simulink model "Impedance_Control"  (R2021b)
settings: Solver=VariableStepAuto  StartTime=0.0  StopTime=10  RelTol=1e-3
undefined symbols (not defined in the file or in its folder): Dm, Km, q_dq_init
(part 2 of 3)

== matlab function Impedance_Control/C ==
  data: q input; C output; dq input
function C = C(q,dq)
%C_fun
%    C = C_fun(Q1,Q2,Q3,Q4,Q5,Q6,DQ1,DQ2,DQ3,DQ4,DQ5,DQ6)

%    This function was generated by the Symbolic Math Toolbox version 9.0.
%    28-Mar-2022 14:37:35

q1 = q(1);
q2 = q(2);
q3 = q(3);
q4 = q(4);
q5 = q(5);
q6 = q(6);

dq1 = dq(1);
dq2 = dq(2);
dq3 = dq(3);
dq4 = dq(4);
dq5 = dq(5);
dq6 = dq(6);

t2 = cos(q1);
t3 = cos(q2);
t4 = cos(q4);
t5 = cos(q5);
t6 = cos(q6);
t7 = sin(q1);
t8 = sin(q2);
t9 = sin(q4);
t10 = sin(q5);
t11 = sin(q6);
t12 = dq1.^2;
t13 = dq2.^2;
t14 = dq4.^2;
t15 = dq5.^2;
t16 = dq6.^2;
t17 = q2.*2.0;
t18 = q3.^2;
t291 = q3-5.6e-3;
t555 = q3-1.56e-2;
t19 = cos(t17);
t20 = t3.^2;
t21 = t4.^2;
t22 = sin(t17);
t23 = t8.^2;
t24 = t9.^2;
t25 = dq2.*t4;
t26 = dq3.*t8;
t27 = dq2.*t9;
t28 = t2.*t4;
t29 = t3.*t5;
t31 = t2.*t9;
t32 = t4.*t7;
t33 = t3.*t10;
t34 = t5.*t8;
t35 = t7.*t9;
t36 = t8.*t10;
t38 = dq1.*t2.*t3;
t40 = dq3.*t2.*t3;
t41 = dq1.*t3.*t4;
t45 = dq4.*t3.*t4;
t47 = dq1.*t3.*t7;
t48 = dq2.*t2.*t8;
t51 = dq3.*t3.*t7;
t52 = dq1.*t3.*t9;
t59 = dq4.*t3.*t9;
t60 = dq4.*t4.*t8;
t63 = dq2.*t7.*t8;
t68 = dq4.*t8.*t9;
t70 = dq2.*dq3.*t3.*2.0;
t74 = t8.*t9.*t11;
t80 = t3.*t4.*t6;
t93 = t3.*t4.*t11;
t94 = t3.*t6.*t9;
t107 = t3.*t9.*t11;
t108 = t6.*t8.*t9;
t250 = t3.*t4.*t13;
t252 = t3.*t4.*t14;
t258 = t3.*t9.*t13;
t262 = t3.*t9.*t14;
t277 = t8.*t13.*1.56e+2;
t574 = dq2.*dq3.*t3.*2.0e+4;
t615 = t2.*t3.*t12.*1.56e+2;
t616 = t2.*t3.*t13.*1.56e+2;
t627 = t3.*t7.*t12.*1.56e+2;
t628 = t3.*t7.*t13.*1.56e+2;
t675 = q3.*t8.*t13.*1.0e+4;
t847 = dq2.*t3.*t291;
t928 = q3.*t2.*t3.*t12.*1.0e+4;
t929 = q3.*t2.*t3.*t13.*1.0e+4;
t935 = q3.*t3.*t7.*t12.*1.0e+4;
t936 = q3.*t3.*t7.*t13.*1.0e+4;
t945 = dq2.*t3.*t555;
t1137 = t8.*t13.*t291;
t1202 = t8.*t13.*t555;
t1234 = t2.*t3.*t12.*t291;
t1235 = t2.*t3.*t13.*t291;
t1241 = t3.*t7.*t12.*t291;
t1242 = t3.*t7.*t13.*t291;
t1250 = t2.*t3.*t12.*t555;
t1251 = t2.*t3.*t13.*t555;
t1255 = t3.*t7.*t12.*t555;
t1256 = t3.*t7.*t13.*t555;
t30 = dq4.*t27;
t37 = dq4.*t25;
t39 = dq1.*t28;
t42 = t3.*t25;
t43 = dq2.*t29;
t44 = dq4.*t28;
t46 = dq5.*t29;
t49 = dq1.*t31;
t50 = dq1.*t32;
t53 = t3.*t27;
t54 = t8.*t25;
t55 = dq2.*t33;
t56 = dq2.*t34;
t57 = dq4.*t31;
t58 = dq4.*t32;
t61 = dq5.*t33;
t62 = dq5.*t34;
t64 = dq1.*t35;
t65 = t8.*t27;
t66 = dq2.*t36;
t67 = dq4.*t35;
t69 = dq5.*t36;
t71 = t8.*t35;
t72 = t7.*t36;
t73 = t10.*t35;
t75 = t11.*t36;
t76 = dq4.*t41;
t77 = t2.*t29;
t78 = t5.*t28;
t79 = t4.*t29;
t81 = t6.*t29;
t83 = dq4.*t52;
t84 = t8.*t28;
t85 = t2.*t33;
t86 = t2.*t34;
t87 = t7.*t29;
t88 = t10.*t28;
t89 = t5.*t31;
t90 = t5.*t32;
t91 = t4.*t33;
t92 = t4.*t34;
t95 = t11.*t29;
t96 = t6.*t34;
t98 = t8.*t31;
t99 = t8.*t32;
t100 = t2.*t36;
t101 = t7.*t33;
t102 = t7.*t34;
t103 = t10.*t31;
t104 = t10.*t32;
t105 = t5.*t35;
t106 = t4.*t36;
t109 = t11.*t34;
t110 = t6.*t36;
t111 = -t70;
t119 = t25.*t29;
t125 = t6.*t45;
t127 = dq6.*t80;
t147 = t25.*t33;
t148 = t25.*t34;
t161 = dq4.*t9.*t29;
t165 = t11.*t45;
t166 = t6.*t59;
t167 = t6.*t60;
t173 = dq6.*t93;
t174 = dq6.*t94;
t195 = t25.*t36;
t196 = t27.*t34;
t208 = dq4.*t9.*t33;
t209 = dq4.*t9.*t34;
t213 = t11.*t59;
t214 = t11.*t60;
t220 = dq6.*t107;
t221 = dq6.*t108;
t224 = -t40;
t233 = t27.*t36;
t237 = dq4.*t9.*t36;
t240 = dq6.*t74;
t242 = -t51;
t243 = -t52;
t244 = -t63;
t248 = -t68;
t249 = t12.*t28;
t251 = t14.*t28;
t253 = dq3.*t38.*2.0;
t256 = t12.*t31;
t257 = t12.*t32;
t259 = t13.*t34;
t260 = t14.*t31;
t261 = t14.*t32;
t263 = t15.*t34;
t264 = dq3.*t47.*2.0;
t265 = dq2.*t2.*t26.*2.0;
t270 = t12.*t35;
t271 = t13.*t36;
t272 = t14.*t35;
t273 = t15.*t36;
t274 = dq2.*t7.*t26.*2.0;
t279 = t38.*1.56e+2;
t280 = t47.*1.56e+2;
t281 = t48.*1.56e+2;
t282 = t63.*1.56e+2;
t283 = t28.*t29;
t285 = t28.*t33;
t286 = t28.*t34;
t287 = t29.*t32;
t288 = t3.*t6.*t31;
t292 = t28.*t36;
t293 = t31.*t34;
t294 = t32.*t33;
t295 = t32.*t34;
t296 = t3.*t11.*t31;
t297 = t3.*t6.*t35;
t299 = t6.*t9.*t33;
t305 = t31.*t36;
t306 = t32.*t36;
t307 = t34.*t35;
t308 = t3.*t11.*t35;
t309 = t9.*t11.*t33;
t315 = -t94;
t316 = t35.*t36;
t323 = -t277;
t466 = t25.*t38.*2.0;
t484 = t13.*t94;
t489 = t14.*t94;
t492 = t16.*t94;
t494 = t27.*t38.*2.0;
t525 = t13.*t107;
t531 = t14.*t107;
t533 = t16.*t107;
t535 = t27.*t47.*2.0;
t570 = dq1.*t48.*3.12e+2;
t573 = dq1.*t63.*3.12e+2;
t576 = dq6.*t6.*t28.*1.0e+2;
t583 = dq6.*t6.*t32.*1.0e+2;
t592 = t40.*1.0e+4;
t595 = t27+t41;
t596 = t51.*1.0e+4;
t634 = -t574;
t782 = dq3.*t38.*2.0e+4;
t787 = q3.*t38.*1.0e+4;
t788 = dq3.*t47.*2.0e+4;
t789 = dq2.*t2.*t26.*2.0e+4;
t790 = q3.*t47.*1.0e+4;
t791 = q3.*t48.*1.0e+4;
t792 = dq2.*t7.*t26.*2.0e+4;
t793 = q3.*t63.*1.0e+4;
t830 = dq1.*q3.*t48.*2.0e+4;
t834 = t47+t48;
t844 = dq1.*q3.*t63.*2.0e+4;
t880 = t11.*t16.*t28.*1.0e+2;
t904 = t11.*t16.*t32.*1.0e+2;
t968 = t11.*t27.*t38.*2.0e+2;
t991 = t11.*t27.*t47.*2.0e+2;
t1030 = t38.*t291;
t1031 = -t928;
t1032 = -t929;
t1035 = t47.*t291;
t1036 = t48.*t291;
t1037 = -t935;
t1038 = -t936;
t1043 = t63.*t291;
t1145 = t38.*t555;
t1148 = t47.*t555;
t1149 = t48.*t555;
t1152 = t63.*t555;
t1248 = t26+t847;
t1287 = -t1250;
t1288 = -t1251;
t1290 = -t1255;
t1291 = -t1256;
t1399 = t25.*1.0e-1;
t1402 = t27.*1.0e-1;
t1412 = t41.*1.0e-1;
t1415 = t52.*1.0e-1;
t82 = dq1.*t54;
t97 = dq1.*t65;
t112 = -t37;
t113 = t3.*t39;
t114 = dq1.*t77;
t115 = t2.*t42;
t116 = t2.*t43;
t117 = t5.*t39;
t118 = t3.*t44;
t120 = t2.*t46;
t121 = t5.*t44;
t122 = t6.*t43;
t123 = dq4.*t79;
t124 = dq5.*t78;
t126 = t4.*t46;
t128 = dq6.*t81;
t129 = t3.*t49;
t130 = t8.*t39;
t131 = t3.*t50;
t132 = dq1.*t85;
t133 = dq1.*t86;
t134 = dq1.*t87;
t135 = t2.*t53;
t136 = t2.*t54;
t137 = t7.*t42;
t138 = t2.*t55;
t139 = t2.*t56;
t140 = t7.*t43;
t141 = t10.*t39;
t142 = t5.*t49;
t143 = t5.*t50;
t144 = t3.*t57;
t145 = t8.*t44;
t146 = t3.*t58;
t149 = t2.*t61;
t150 = t2.*t62;
t151 = t7.*t46;
t152 = t6.*t53;
t153 = t6.*t54;
t154 = t10.*t44;
t155 = t5.*t57;
t156 = t5.*t58;
t157 = t11.*t43;
t158 = t6.*t55;
t159 = t6.*t56;
t160 = dq4.*t91;
t162 = dq5.*t88;
t163 = dq5.*t89;
t164 = dq5.*t90;
t168 = t4.*t61;
t169 = t9.*t46;
t170 = t4.*t62;
t171 = t6.*t61;
t172 = t6.*t62;
t175 = dq6.*t95;
t176 = dq6.*t96;
t177 = t8.*t49;
t178 = t3.*t64;
t179 = t8.*t50;
t180 = dq1.*t100;
t181 = dq1.*t101;
t182 = dq1.*t102;
t183 = t2.*t65;
t184 = t7.*t53;
t185 = t7.*t54;
t186 = t2.*t66;
t187 = t7.*t55;
t188 = t7.*t56;
t189 = t10.*t49;
t190 = t10.*t50;
t191 = t5.*t64;
t192 = t8.*t57;
t193 = t3.*t67;
t194 = t8.*t58;
t197 = t2.*t69;
t198 = t7.*t61;
t199 = t7.*t62;
t200 = t11.*t53;
t201 = t11.*t54;
t202 = t6.*t65;
t203 = t10.*t57;
t204 = t10.*t58;
t205 = t5.*t67;
t206 = t11.*t55;
t207 = t11.*t56;
t210 = dq5.*t103;
t211 = dq5.*t104;
t212 = dq5.*t105;
t215 = t9.*t61;
t216 = t4.*t69;
t217 = t11.*t61;
t218 = t11.*t62;
t219 = t6.*t69;
t222 = dq6.*t109;
t223 = dq6.*t110;
t225 = -t43;
t226 = -t46;
t227 = t8.*t64;
t228 = dq1.*t72;
t229 = t7.*t65;
t230 = t7.*t66;
t231 = t10.*t64;
t232 = t8.*t67;
t234 = t7.*t69;
t235 = t11.*t65;
t236 = t10.*t67;
t238 = dq5.*t73;
t239 = t11.*t69;
t241 = dq6.*t75;
t245 = -t64;
t246 = -t65;
t247 = -t67;
t254 = dq4.*t39.*2.0;
t255 = dq5.*t43.*2.0;
t266 = dq4.*t49.*2.0;
t267 = dq4.*t50.*2.0;
t268 = t8.*t37.*2.0;
t269 = dq5.*t55.*2.0;
t275 = dq4.*t64.*2.0;
t276 = t8.*t30.*2.0;
t278 = -t71;
t284 = t6.*t79;
t289 = t11.*t79;
t290 = t6.*t91;
t298 = t11.*t91;
t300 = t6.*t106;
t301 = -t253;
t303 = -t79;
t304 = -t81;
t310 = t4.*t75;
t311 = -t264;
t312 = -t265;
t313 = -t84;
t314 = -t87;
t318 = -t274;
t321 = -t105;
t322 = -t106;
t324 = t29.*t39;
t325 = t25.*t77;
t327 = t28.*t46;
t330 = t33.*t39;
t331 = t34.*t39;
t332 = t29.*t50;
t334 = t25.*t85;
t335 = t27.*t77;
t336 = t25.*t86;
t337 = t25.*t87;
t338 = t29.*t57;
t339 = t34.*t44;
t342 = t28.*t61;
t343 = t28.*t62;
t344 = t32.*t46;
t345 = t6.*t147;
t346 = t25.*t96;
t347 = dq6.*t288;
t349 = dq4.*t9.*t81;
t356 = t36.*t39;
t357 = t34.*t49;
t358 = t33.*t50;
t359 = t34.*t50;
t362 = t27.*t85;
t363 = t25.*t100;
t364 = t25.*t101;
t365 = t27.*t87;
t366 = t25.*t102;
t368 = t33.*t57;
t369 = t36.*t44;
t370 = t34.*t57;
t371 = t29.*t67;
t372 = t34.*t58;
t374 = t28.*t69;
t375 = t31.*t62;
t376 = t32.*t61;
t377 = t32.*t62;
t378 = t11.*t147;
t379 = t25.*t109;
t380 = t25.*t110;
t381 = dq6.*t296;
t382 = dq6.*t297;
t384 = dq4.*t9.*t95;
t385 = t6.*t208;
t390 = dq6.*t299;
t398 = -t119;
t403 = -t125;
t405 = -t127;
t407 = t36.*t49;
t408 = t36.*t50;
t409 = t34.*t64;
t411 = t27.*t101;
t412 = t25.*t72;
t415 = t36.*t57;
t416 = t33.*t67;
t417 = t36.*t58;
t418 = t34.*t67;
t419 = t31.*t69;
t420 = t32.*t69;
t421 = t35.*t62;
t422 = t25.*t75;
t423 = t27.*t110;
t424 = dq6.*t308;
t425 = t11.*t208;
t426 = dq4.*t9.*t110;
t427 = dq6.*t309;
t430 = -t165;
t431 = -t167;
t432 = -t174;
t433 = t36.*t64;
t435 = t36.*t67;
t436 = t35.*t69;
t437 = t27.*t75;
t438 = dq4.*t9.*t75;
t450 = -t233;
t453 = -t237;
t457 = -t280;
t458 = -t281;
t459 = -t282;
t460 = t12.*t77;
t461 = t13.*t77;
t462 = t13.*t79;
t463 = t15.*t77;
t464 = t14.*t79;
t465 = t15.*t79;
t467 = t2.*t3.*t37.*2.0;
t472 = dq6.*t125.*2.0;
t473 = t12.*t84;
t474 = t12.*t85;
t475 = t12.*t87;
t476 = t13.*t84;
t477 = t13.*t85;
t478 = t13.*t87;
t479 = t12.*t89;
t480 = t14.*t84;
t481 = t13.*t91;
t482 = t15.*t85;
t483 = t15.*t87;
t485 = t14.*t89;
t486 = t13.*t96;
t487 = t14.*t91;
t488 = t15.*t89;
t490 = t15.*t91;
t491 = t15.*t96;
t493 = t16.*t96;
t498 = t2.*t3.*t30.*2.0;
C = ft_1({dq1,dq2,dq3,dq4,dq5,dq6,q3,t10,t100,t101,t102,t103,t1030,t1031,t1032,t1035,t1036,t1037,t1038,t104,t1043,t105,t106,t107,t108,t109,t11,t110,t111,t112,t113,t1137,t114,t1145,t1148,t1149,t115,t1152,t116,t117,t118,t12,t120,t1202,t121,t122,t123,t1234,t1235,t124,t1241,t1242,t1248,t125,t126,t128,t1287,t1288,t129,t1290,t1291,t13,t130,t131,t132,t133,t134,t135,t136,t137,t138,t139,t1399,t14,t140,t1402,t141,t1412,t1415,t142,t143,t144,t145,t146,t147,t148,t149,t15,t150,t151,t152,t153,t154,t155,t156,t157,t158,t159,t16,t160,t161,t162,t163,t164,t165,t166,t168,t169,t170,t171,t172,t173,t175,t176,t177,t178,t179,t18,t180,t181,t182,t183,t184,t185,t186,t187,t188,t189,t19,t190,t191,t192,t193,t194,t195,t196,t197,t198,t199,t2,t20,t200,t201,t202,t203,t204,t205,t206,t207,t208,t209,t21,t210,t211,t212,t213,t214,t215,t216,t217,t218,t219,t22,t220,t221,t222,t223,t224,t225,t226,t227,t228,t229,t23,t230,t231,t232,t233,t234,t235,t236,t238,t239,t24,t240,t241,t242,t243,t244,t245,t246,t247,t248,t249,t25,t250,t251,t252,t253,t254,t255,t256,t257,t258,t259,t26,t260,t261,t262,t263,t264,t265,t266,t267,t268,t269,t270,t271,t272,t273,t274,t275,t276,t278,t279,t28,t283,t284,t285,t286,t287,t288,t289,t29,t290,t291,t292,t293,t294,t295,t296,t297,t298,t299,t3,t30,t300,t301,t303,t304,t305,t306,t307,t308,t309,t31,t310,t311,t312,t313,t314,t315,t316,t318,t32,t321,t322,t323,t324,t325,t33,t330,t331,t332,t334,t335,t336,t337,t338,t339,t34,t342,t343,t344,t345,t346,t347,t349,t35,t356,t357,t358,t359,t36,t362,t363,t364,t365,t366,t368,t369,t37,t370,t371,t372,t374,t375,t376,t377,t378,t379,t38,t380,t381,t382,t384,t385,t39,t390,t398,t4,t40,t403,t405,t407,t408,t409,t411,t412,t415,t417,t419,t42,t420,t421,t422,t423,t424,t425,t426,t427,t43,t430,t431,t432,t433,t435,t436,t437,t438,t44,t45,t450,t453,t457,t458,t459,t460,t461,t463,t466,t467,t47,t472,t473,t474,t475,t476,t477,t478,t479,t48,t480,t481,t482,t483,t485,t486,t487,t488,t49,t490,t491,t493,t494,t498,t5,t50,t51,t525,t53,t531,t533,t535,t54,t55,t555,t56,t57,t570,t573,t576,t58,t583,t59,t592,t595,t596,t6,t60,t61,t615,t616,t62,t627,t628,t63,t634,t64,t65,t66,t67,t675,t69,t7,t70,t71,t72,t73,t74,t75,t76,t77,t78,t782,t787,t788,t789,t79,t790,t791,t792,t793,t8,t80,t81,t82,t83,t830,t834,t84,t844,t847,t85,t86,t87,t88,t880,t89,t9,t90,t904,t91,t92,t93,t94,t945,t95,t96,t968,t97,t98,t99,t991});
end
function C = ft_1(ct)
dq1 = ct{1};
dq2 = ct{2};
dq3 = ct{3};
dq4 = ct{4};
dq5 = ct{5};
dq6 = ct{6};
q3 = ct{7};
t10 = ct{8};
t100 = ct{9};
t101 = ct{10};
t102 = ct{11};
t103 = ct{12};
t1030 = ct{13};
t1031 = ct{14};
t1032 = ct{15};
t1035 = ct{16};
t1036 = ct{17};
t1037 = ct{18};
t1038 = ct{19};
t104 = ct{20};
t1043 = ct{21};
t105 = ct{22};
t106 = ct{23};
t107 = ct{24};
t108 = ct{25};
t109 = ct{26};
t11 = ct{27};
t110 = ct{28};
t111 = ct{29};
t112 = ct{30};
t113 = ct{31};
t1137 = ct{32};
t114 = ct{33};
t1145 = ct{34};
t1148 = ct{35};
t1149 = ct{36};
t115 = ct{37};
t1152 = ct{38};
t116 = ct{39};
t117 = ct{40};
t118 = ct{41};
t12 = ct{42};
t120 = ct{43};
t1202 = ct{44};
t121 = ct{45};
t122 = ct{46};
t123 = ct{47};
t1234 = ct{48};
t1235 = ct{49};
t124 = ct{50};
t1241 = ct{51};
t1242 = ct{52};
t1248 = ct{53};
t125 = ct{54};
t126 = ct{55};
t128 = ct{56};
t1287 = ct{57};
t1288 = ct{58};
t129 = ct{59};
t1290 = ct{60};
t1291 = ct{61};
t13 = ct{62};
t130 = ct{63};
t131 = ct{64};
t132 = ct{65};
t133 = ct{66};
t134 = ct{67};
t135 = ct{68};
t136 = ct{69};
t137 = ct{70};
t138 = ct{71};
t139 = ct{72};
t1399 = ct{73};
t14 = ct{74};
t140 = ct{75};
t1402 = ct{76};
t141 = ct{77};
t1412 = ct{78};
t1415 = ct{79};
t142 = ct{80};
t143 = ct{81};
t144 = ct{82};
t145 = ct{83};
t146 = ct{84};
t147 = ct{85};
t148 = ct{86};
t149 = ct{87};
t15 = ct{88};
t150 = ct{89};
t151 = ct{90};
t152 = ct{91};
t153 = ct{92};
t154 = ct{93};
t155 = ct{94};
t156 = ct{95};
t157 = ct{96};
t158 = ct{97};
t159 = ct{98};
t16 = ct{99};
t160 = ct{100};
t161 = ct{101};
t162 = ct{102};
t163 = ct{103};
t164 = ct{104};
t165 = ct{105};
t166 = ct{106};
t168 = ct{107};
t169 = ct{108};
t170 = ct{109};
t171 = ct{110};
t172 = ct{111};
t173 = ct{112};
t175 = ct{113};
t176 = ct{114};
t177 = ct{115};
t178 = ct{116};
t179 = ct{117};
t18 = ct{118};
t180 = ct{119};
t181 = ct{120};
t182 = ct{121};
t183 = ct{122};
t184 = ct{123};
t185 = ct{124};
t186 = ct{125};
t187 = ct{126};
t188 = ct{127};
t189 = ct{128};
t19 = ct{129};
t190 = ct{130};
t191 = ct{131};
t192 = ct{132};
t193 = ct{133};
t194 = ct{134};
t195 = ct{135};
t196 = ct{136};
t197 = ct{137};
t198 = ct{138};
t199 = ct{139};
t2 = ct{140};
t20 = ct{141};
t200 = ct{142};
t201 = ct{143};
t202 = ct{144};
t203 = ct{145};
t204 = ct{146};
t205 = ct{147};
t206 = ct{148};
t207 = ct{149};
t208 = ct{150};
t209 = ct{151};
t21 = ct{152};
t210 = ct{153};
t211 = ct{154};
t212 = ct{155};
t213 = ct{156};
t214 = ct{157};
t215 = ct{158};
t216 = ct{159};
t217 = ct{160};
t218 = ct{161};
t219 = ct{162};
t22 = ct{163};
t220 = ct{164};
t221 = ct{165};
t222 = ct{166};
t223 = ct{167};
t224 = ct{168};
t225 = ct{169};
t226 = ct{170};
t227 = ct{171};
t228 = ct{172};
t229 = ct{173};
t23 = ct{174};
t230 = ct{175};
t231 = ct{176};
t232 = ct{177};
t233 = ct{178};
t234 = ct{179};
t235 = ct{180};
t236 = ct{181};
t238 = ct{182};
t239 = ct{183};
t24 = ct{184};
t240 = ct{185};
t241 = ct{186};
t242 = ct{187};
t243 = ct{188};
t244 = ct{189};
t245 = ct{190};
t246 = ct{191};
t247 = ct{192};
t248 = ct{193};
t249 = ct{194};
t25 = ct{195};
t250 = ct{196};
t251 = ct{197};
t252 = ct{198};
t253 = ct{199};
t254 = ct{200};
t255 = ct{201};
t256 = ct{202};
t257 = ct{203};
t258 = ct{204};
t259 = ct{205};
t26 = ct{206};
t260 = ct{207};
t261 = ct{208};
t262 = ct{209};
t263 = ct{210};
t264 = ct{211};
t265 = ct{212};
t266 = ct{213};
t267 = ct{214};
t268 = ct{215};
t269 = ct{216};
t270 = ct{217};
t271 = ct{218};
t272 = ct{219};
t273 = ct{220};
t274 = ct{221};
t275 = ct{222};
t276 = ct{223};
t278 = ct{224};
t279 = ct{225};
t28 = ct{226};
t283 = ct{227};
t284 = ct{228};
t285 = ct{229};
t286 = ct{230};
t287 = ct{231};
t288 = ct{232};
t289 = ct{233};
t29 = ct{234};
t290 = ct{235};
t291 = ct{236};
t292 = ct{237};
t293 = ct{238};
t294 = ct{239};
t295 = ct{240};
t296 = ct{241};
t297 = ct{242};
t298 = ct{243};
t299 = ct{244};
t3 = ct{245};
t30 = ct{246};
t300 = ct{247};
t301 = ct{248};
t303 = ct{249};
t304 = ct{250};
t305 = ct{251};
t306 = ct{252};
t307 = ct{253};
t308 = ct{254};
t309 = ct{255};
t31 = ct{256};
t310 = ct{257};
t311 = ct{258};
t312 = ct{259};
t313 = ct{260};
t314 = ct{261};
t315 = ct{262};
t316 = ct{263};
t318 = ct{264};
t32 = ct{265};
t321 = ct{266};
t322 = ct{267};
t323 = ct{268};
t324 = ct{269};
t325 = ct{270};
t33 = ct{271};
t330 = ct{272};
t331 = ct{273};
t332 = ct{274};
t334 = ct{275};
t335 = ct{276};
t336 = ct{277};
t337 = ct{278};
t338 = ct{279};
t339 = ct{280};
t34 = ct{281};
t342 = ct{282};
t343 = ct{283};
t344 = ct{284};
t345 = ct{285};
t346 = ct{286};
t347 = ct{287};
t349 = ct{288};
t35 = ct{289};
t356 = ct{290};
t357 = ct{291};
t358 = ct{292};
t359 = ct{293};
t36 = ct{294};
t362 = ct{295};
t363 = ct{296};
t364 = ct{297};
t365 = ct{298};
t366 = ct{299};
t368 = ct{300};
t369 = ct{301};
t37 = ct{302};
t370 = ct{303};
t371 = ct{304};
t372 = ct{305};
t374 = ct{306};
t375 = ct{307};
t376 = ct{308};
t377 = ct{309};
t378 = ct{310};
t379 = ct{311};
t38 = ct{312};
t380 = ct{313};
t381 = ct{314};
t382 = ct{315};
t384 = ct{316};
t385 = ct{317};
t39 = ct{318};
t390 = ct{319};
t398 = ct{320};
t4 = ct{321};
t40 = ct{322};
t403 = ct{323};
t405 = ct{324};
t407 = ct{325};
t408 = ct{326};
t409 = ct{327};
t411 = ct{328};
t412 = ct{329};
t415 = ct{330};
t417 = ct{331};
t419 = ct{332};
t42 = ct{333};
t420 = ct{334};
t421 = ct{335};
t422 = ct{336};
t423 = ct{337};
t424 = ct{338};
t425 = ct{339};
t426 = ct{340};
t427 = ct{341};
t43 = ct{342};
t430 = ct{343};
t431 = ct{344};
t432 = ct{345};
t433 = ct{346};
t435 = ct{347};
t436 = ct{348};
t437 = ct{349};
t438 = ct{350};
t44 = ct{351};
t45 = ct{352};
t450 = ct{353};
t453 = ct{354};
t457 = ct{355};
t458 = ct{356};
t459 = ct{357};
t460 = ct{358};
t461 = ct{359};
t463 = ct{360};
t466 = ct{361};
t467 = ct{362};
t47 = ct{363};
t472 = ct{364};
t473 = ct{365};
t474 = ct{366};
t475 = ct{367};
t476 = ct{368};
t477 = ct{369};
t478 = ct{370};
t479 = ct{371};
t48 = ct{372};
t480 = ct{373};
t481 = ct{374};
t482 = ct{375};
t483 = ct{376};
t485 = ct{377};
t486 = ct{378};
t487 = ct{379};
t488 = ct{380};
t49 = ct{381};
t490 = ct{382};
t491 = ct{383};
t493 = ct{384};
t494 = ct{385};
t498 = ct{386};
t5 = ct{387};
t50 = ct{388};
t51 = ct{389};
t525 = ct{390};
t53 = ct{391};
t531 = ct{392};
t533 = ct{393};
t535 = ct{394};
t54 = ct{395};
t55 = ct{396};
t555 = ct{397};
t56 = ct{398};
t57 = ct{399};
t570 = ct{400};
t573 = ct{401};
t576 = ct{402};
t58 = ct{403};
t583 = ct{404};
t59 = ct{405};
t592 = ct{406};
t595 = ct{407};
t596 = ct{408};
t6 = ct{409};
t60 = ct{410};
t61 = ct{411};
t615 = ct{412};
t616 = ct{413};
t62 = ct{414};
t627 = ct{415};
t628 = ct{416};
t63 = ct{417};
t634 = ct{418};
t64 = ct{419};
t65 = ct{420};
t66 = ct{421};
t67 = ct{422};
t675 = ct{423};
t69 = ct{424};
t7 = ct{425};
t70 = ct{426};
t71 = ct{427};
t72 = ct{428};
t73 = ct{429};
t74 = ct{430};
t75 = ct{431};
t76 = ct{432};
t77 = ct{433};
t78 = ct{434};
t782 = ct{435};
t787 = ct{436};
t788 = ct{437};
t789 = ct{438};
t79 = ct{439};
t790 = ct{440};
t791 = ct{441};
t792 = ct{442};
t793 = ct{443};
t8 = ct{444};
t80 = ct{445};
t81 = ct{446};
t82 = ct{447};
t83 = ct{448};
t830 = ct{449};
t834 = ct{450};
t84 = ct{451};
t844 = ct{452};
t847 = ct{453};
t85 = ct{454};
t86 = ct{455};
t87 = ct{456};
t88 = ct{457};
t880 = ct{458};
t89 = ct{459};
t9 = ct{460};
t90 = ct{461};
t904 = ct{462};
t91 = ct{463};
t92 = ct{464};
t93 = ct{465};
t94 = ct{466};
t945 = ct{467};
t95 = ct{468};
t96 = ct{469};
t968 = ct{470};
t97 = ct{471};
t98 = ct{472};
t99 = ct{473};
t991 = ct{474};
t499 = t3.*t7.*t37.*2.0;
t507 = t25.*t62.*2.0;
t513 = dq6.*t165.*2.0;
t514 = t12.*t98;
t515 = t12.*t99;
t516 = t12.*t101;
t517 = t13.*t98;
t518 = t13.*t99;
t519 = t13.*t101;
t520 = t12.*t103;
t521 = t12.*t105;
t522 = t14.*t98;
t523 = t14.*t99;
t524 = t15.*t101;
t526 = t14.*t103;
t527 = t14.*t105;
t528 = t13.*t109;
t529 = t15.*t103;
t530 = t15.*t105;
t532 = t15.*t109;
t534 = t16.*t109;
t540 = t3.*t7.*t30.*2.0;
t547 = t30.*t34.*2.0;
t549 = t25.*t69.*2.0;
t556 = t12.*t71;
t557 = t13.*t71;
t558 = t12.*t73;
t559 = t14.*t71;
t560 = t14.*t73;
t561 = t15.*t73;
t566 = t30.*t36.*2.0;
t569 = dq5.*t55.*1.82e+2;
t571 = -t270;
t572 = -t272;
t582 = t11.*t39.*1.0e+2;
t589 = t11.*t50.*1.0e+2;
t590 = t11.*t57.*1.0e+2;
t591 = t43./1.0e+2;
t594 = t11.*t67.*1.0e+2;
t597 = t69./1.0e+2;
t598 = -t466;
t604 = -t283;
t608 = t6.*t8.*t37.*-2.0;
t610 = -t287;
t611 = -t288;
t617 = -t292;
t618 = -t297;
t619 = -t299;
t625 = t259.*9.1e+1;
t626 = t263.*9.1e+1;
t629 = -t307;
t631 = (dq5.*t55)./5.0e+1;
t632 = -t316;
t633 = -t573;
t651 = -t576;
t672 = -t592;
t679 = -t596;
t680 = t34.*t249;
t681 = t28.*t259;
t682 = t34.*t251;
t683 = t28.*t263;
t690 = t39.*t62.*2.0;
t691 = t30.*t77.*2.0;
t698 = t36.*t249;
t699 = t34.*t257;
t700 = t28.*t271;
t701 = t32.*t259;
t702 = t36.*t251;
t703 = t34.*t261;
t704 = t28.*t273;
t705 = t32.*t263;
t712 = t39.*t69.*2.0;
t713 = t50.*t62.*2.0;
t714 = t30.*t85.*2.0;
t715 = t30.*t87.*2.0;
t717 = t57.*t62.*2.0;
t728 = t36.*t257;
t729 = t32.*t271;
t730 = t36.*t261;
t731 = t32.*t273;
t733 = dq6.*t6.*t39.*2.0e+2;
t734 = dq6.*t125.*2.0e+2;
t737 = t50.*t69.*2.0;
t738 = t30.*t101.*2.0;
t739 = t57.*t69.*2.0;
t740 = t62.*t67.*2.0;
t741 = t30.*t110.*2.0;
t747 = t13.*t315;
t748 = t14.*t315;
t749 = t16.*t315;
t754 = t25.*t62.*1.82e+2;
t757 = dq6.*t6.*t50.*2.0e+2;
t760 = dq6.*t6.*t57.*2.0e+2;
t762 = t67.*t69.*2.0;
t763 = t30.*t75.*2.0;
t772 = dq4.*t11.*t49.*2.0e+2;
t773 = t8.*t11.*t37.*2.0e+2;
t775 = dq6.*t6.*t67.*2.0e+2;
t784 = t30.*t36.*1.82e+2;
t785 = dq4.*t11.*t64.*2.0e+2;
t797 = dq1.*t7.*t81.*1.0e+2;
t801 = dq6.*t11.*t77.*1.0e+2;
t811 = dq6.*t6.*t98.*1.0e+2;
t813 = dq6.*t11.*t87.*1.0e+2;
t823 = dq6.*t6.*t71.*1.0e+2;
t824 = dq6.*t11.*t103.*1.0e+2;
t833 = dq6.*t11.*t73.*1.0e+2;
t835 = t53+t60;
t836 = t54+t59;
t839 = t195./1.0e+2;
t842 = t208./1.0e+2;
t845 = t33+t92;
t846 = t34+t91;
t849 = t31+t99;
t850 = t32+t98;
t851 = t25+t243;
t877 = t11.*t249.*1.0e+2;
t879 = t11.*t251.*1.0e+2;
t887 = (t25.*t62)./5.0e+1;
t900 = t11.*t257.*1.0e+2;
t901 = t525.*1.0e+2;
t902 = t11.*t261.*1.0e+2;
t903 = t531.*1.0e+2;
t905 = t533.*1.0e+2;
t915 = (t30.*t36)./5.0e+1;
t918 = t259./1.0e+2;
t919 = t263./1.0e+2;
t920 = -t787;
t921 = -t788;
t922 = -t789;
t923 = -t792;
t937 = -t830;
t950 = t39.*t62.*1.82e+2;
t953 = t2.*t3.*t11.*t37.*2.0e+2;
t965 = t50.*t62.*1.82e+2;
t966 = t30.*t85.*1.82e+2;
t967 = t57.*t62.*1.82e+2;
t971 = t3.*t7.*t11.*t37.*2.0e+2;
t989 = t30.*t101.*1.82e+2;
t990 = t62.*t67.*1.82e+2;
t997 = t30.*t110.*2.0e+2;
t1008 = -t880;
t1017 = t39.*t110.*1.0e+2;
t1020 = t50.*t110.*1.0e+2;
t1021 = t57.*t110.*1.0e+2;
t1025 = t67.*t110.*1.0e+2;
t1040 = t38+t244;
t1041 = t42+t248;
t1051 = t6.*t16.*t77.*1.0e+2;
t1055 = t7.*t12.*t81.*1.0e+2;
t1056 = t7.*t13.*t81.*1.0e+2;
t1058 = t7.*t15.*t81.*1.0e+2;
t1059 = t7.*t16.*t81.*1.0e+2;
t1064 = (t39.*t62)./5.0e+1;
t1082 = t6.*t16.*t103.*1.0e+2;
t1084 = (t50.*t62)./5.0e+1;
t1085 = (t30.*t85)./5.0e+1;
t1086 = (t57.*t62)./5.0e+1;
t1087 = -t968;
t1104 = t11.*t16.*t98.*1.0e+2;
t1107 = t6.*t16.*t73.*1.0e+2;
t1109 = (t30.*t101)./5.0e+1;
t1110 = (t62.*t67)./5.0e+1;
t1126 = t11.*t16.*t71.*1.0e+2;
t1158 = t6.*t30.*t85.*2.0e+2;
t1167 = dq4.*t49.*t110.*2.0e+2;
t1168 = t6.*t30.*t101.*2.0e+2;
t1180 = dq4.*t64.*t110.*2.0e+2;
t1205 = t86+t285;
t1208 = t90+t293;
t1209 = t80+t309;
t1210 = t102+t294;
t1211 = t104+t305;
t1213 = t244.*t291;
t1217 = t110.*t249.*1.0e+2;
t1218 = t13.*t28.*t110.*1.0e+2;
t1219 = t110.*t251.*1.0e+2;
t1220 = t15.*t28.*t110.*1.0e+2;
t1221 = t16.*t28.*t110.*1.0e+2;
t1222 = t110.*t257.*1.0e+2;
t1223 = t13.*t32.*t110.*1.0e+2;
t1224 = t110.*t261.*1.0e+2;
t1225 = t15.*t32.*t110.*1.0e+2;
t1226 = t16.*t32.*t110.*1.0e+2;
t1243 = dq1.*t1036.*2.0;
t1244 = dq1.*t1043.*2.0;
t1247 = -t1145;
t1257 = dq1.*t1149.*2.0;
t1262 = dq1.*t1152.*2.0;
t1308 = t111+t1137;
t1317 = t89+t101+t295;
t1374 = t224+t1035+t1036;
t1405 = t30.*1.0e-1;
t1407 = t37.*1.0e-1;
t1420 = -t1415;
t1422 = t76.*1.0e-1;
t1425 = t83.*1.0e-1;
t1511 = t1402+t1412;
t302 = -t255;
t317 = -t97;
t319 = -t275;
t320 = -t276;
t326 = t6.*t118;
t328 = t6.*t126;
t329 = dq6.*t284;
t333 = t6.*t129;
t340 = t11.*t118;
t341 = t6.*t146;
t348 = t6.*t160;
t350 = t11.*t126;
t351 = t6.*t168;
t352 = t6.*t169;
t353 = t6.*t170;
t354 = dq6.*t289;
t355 = dq6.*t290;
t360 = t11.*t129;
t361 = t6.*t178;
t367 = t6.*t183;
t373 = t11.*t146;
t383 = t11.*t160;
t386 = t11.*t168;
t387 = t11.*t169;
t388 = t11.*t170;
t389 = dq6.*t298;
t391 = dq6.*t300;
t392 = -t113;
t393 = -t114;
t394 = -t115;
t395 = -t116;
t396 = -t117;
t397 = -t118;
t399 = -t120;
t400 = -t122;
t401 = -t123;
t402 = -t124;
t404 = -t126;
t406 = -t128;
t410 = t11.*t178;
t413 = t11.*t183;
t414 = t7.*t202;
t428 = t4.*t241;
t429 = -t152;
t434 = t11.*t229;
t439 = -t189;
t440 = -t191;
t441 = -t204;
t442 = -t210;
t443 = -t212;
t444 = -t227;
t445 = -t228;
t446 = -t229;
t447 = -t230;
t448 = -t231;
t449 = -t232;
t451 = -t234;
t452 = -t236;
t454 = -t238;
t455 = -t239;
t456 = -t241;
t468 = dq1.*t120.*2.0;
t469 = dq4.*t117.*2.0;
t470 = dq5.*t121.*2.0;
t471 = dq6.*t122.*2.0;
t495 = dq1.*t137.*2.0;
t496 = dq1.*t139.*2.0;
t497 = dq4.*t130.*2.0;
t500 = dq1.*t149.*2.0;
t501 = dq1.*t151.*2.0;
t502 = dq4.*t141.*2.0;
t503 = dq4.*t143.*2.0;
t504 = dq5.*t139.*2.0;
t505 = dq5.*t142.*2.0;
t506 = t6.*t268;
t508 = dq5.*t154.*2.0;
t509 = dq5.*t156.*2.0;
t510 = dq5.*t158.*2.0;
t511 = dq4.*t169.*2.0;
t512 = dq6.*t157.*2.0;
t536 = dq1.*t186.*2.0;
t537 = dq1.*t188.*2.0;
t538 = dq4.*t177.*2.0;
t539 = dq4.*t179.*2.0;
t541 = dq1.*t198.*2.0;
t542 = dq4.*t190.*2.0;
t543 = dq5.*t186.*2.0;
t544 = dq5.*t188.*2.0;
t545 = dq5.*t189.*2.0;
t546 = dq5.*t191.*2.0;
t548 = t11.*t268;
t550 = dq5.*t204.*2.0;
t551 = dq5.*t206.*2.0;
t552 = dq6.*t202.*2.0;
t553 = dq4.*t215.*2.0;
t554 = dq6.*t219.*2.0;
t562 = dq1.*t230.*2.0;
t563 = dq4.*t227.*2.0;
t564 = dq5.*t230.*2.0;
t565 = dq5.*t231.*2.0;
t567 = dq6.*t235.*2.0;
t568 = dq6.*t239.*2.0;
t575 = t114.*9.1e+1;
t577 = t134.*9.1e+1;
t578 = t139.*9.1e+1;
t579 = t149.*9.1e+1;
t580 = t154.*9.1e+1;
t581 = t163.*9.1e+1;
t584 = t188.*9.1e+1;
t585 = t189.*9.1e+1;
t586 = t198.*9.1e+1;
t587 = t204.*9.1e+1;
t588 = t212.*9.1e+1;
t593 = t231.*9.1e+1;
t599 = -t467;
t603 = -t472;
t605 = -t284;
t609 = -t513;
t612 = -t289;
t623 = -t566;
t630 = -t310;
t635 = -t324;
t636 = -t325;
t638 = t28.*t226;
t642 = -t335;
t643 = -t339;
t646 = -t347;
t649 = -t390;
t652 = -t408;
t653 = -t412;
t654 = -t415;
t655 = t33.*t247;
t656 = t34.*t247;
t657 = -t420;
t658 = -t422;
t659 = -t423;
t660 = -t425;
t661 = -t426;
t662 = -t427;
t664 = t36.*t245;
t666 = t36.*t247;
t667 = -t436;
t668 = -t438;
t674 = -t594;
t676 = t25.*t114.*2.0;
t677 = t25.*t120.*2.0;
t684 = t13.*t290;
t685 = t14.*t290;
t686 = t15.*t290;
t687 = t16.*t290;
t688 = t25.*t132.*2.0;
t689 = t25.*t134.*2.0;
t692 = t25.*t149.*2.0;
t693 = t25.*t151.*2.0;
t694 = t25.*t172.*2.0;
t697 = -t597;
t706 = t13.*t298;
t707 = t14.*t298;
t708 = t15.*t298;
t709 = t16.*t298;
t710 = t25.*t181.*2.0;
t711 = t34.*t266;
t716 = t25.*t198.*2.0;
t718 = t25.*t218.*2.0;
t719 = t25.*t223.*2.0;
t721 = dq6.*t385.*2.0;
t722 = -t460;
t723 = -t461;
t724 = t13.*t303;
t725 = -t463;
t726 = t14.*t303;
t727 = t15.*t303;
t732 = dq5.*t121.*1.82e+2;
t735 = t36.*t266;
t736 = t34.*t275;
t742 = t25.*t241.*2.0;
t743 = dq6.*t425.*2.0;
t744 = t12.*t314;
t745 = t13.*t314;
t746 = t15.*t314;
t750 = dq1.*t139.*1.82e+2;
t751 = dq1.*t149.*1.82e+2;
t752 = dq4.*t141.*1.82e+2;
t753 = dq5.*t142.*1.82e+2;
t755 = dq5.*t156.*1.82e+2;
t756 = dq4.*t169.*1.82e+2;
t758 = dq5.*t158.*2.0e+2;
t759 = dq6.*t157.*2.0e+2;
t761 = t36.*t275;
t764 = t12.*t321;
t765 = t14.*t321;
t766 = t15.*t321;
t767 = dq1.*t188.*1.82e+2;
t768 = dq1.*t198.*1.82e+2;
t769 = dq4.*t190.*1.82e+2;
t770 = dq5.*t186.*1.82e+2;
t771 = dq5.*t191.*1.82e+2;
t774 = dq6.*t202.*2.0e+2;
t776 = t12.*t278;
t777 = t13.*t278;
t778 = -t558;
t779 = t14.*t278;
t780 = -t560;
t781 = -t561;
t783 = dq5.*t230.*1.82e+2;
t786 = dq6.*t239.*2.0e+2;
t794 = t6.*t114.*1.0e+2;
t795 = t334.*9.1e+1;
t796 = t343.*9.1e+1;
t798 = t6.*t139.*1.0e+2;
t799 = t6.*t149.*1.0e+2;
t800 = t6.*t154.*1.0e+2;
t802 = t6.*t163.*1.0e+2;
t803 = t356.*9.1e+1;
t804 = t364.*9.1e+1;
t805 = t377.*9.1e+1;
t806 = t11.*t135.*1.0e+2;
t807 = t7.*t159.*1.0e+2;
t808 = t6.*t189.*1.0e+2;
t809 = t11.*t145.*1.0e+2;
t810 = t7.*t171.*1.0e+2;
t812 = t6.*t204.*1.0e+2;
t814 = t6.*t212.*1.0e+2;
t815 = t114./1.0e+2;
t816 = t126./1.0e+2;
t817 = t408.*9.1e+1;
t818 = t415.*9.1e+1;
t819 = t11.*t177.*1.0e+2;
t820 = t11.*t184.*1.0e+2;
t821 = t6.*t231.*1.0e+2;
t822 = t11.*t194.*1.0e+2;
t825 = t134./1.0e+2;
t826 = t139./1.0e+2;
t827 = t149./1.0e+2;
t828 = t154./1.0e+2;
t829 = t163./1.0e+2;
t831 = t435.*9.1e+1;
t832 = t11.*t227.*1.0e+2;
t837 = t188./1.0e+2;
t838 = t189./1.0e+2;
t840 = t198./1.0e+2;
t841 = t204./1.0e+2;
t843 = t212./1.0e+2;
t848 = t231./1.0e+2;
t856 = -t690;
t858 = t460.*9.1e+1;
t859 = t461.*9.1e+1;
t860 = t463.*9.1e+1;
t861 = (dq5.*t121)./5.0e+1;
t863 = -t733;
t864 = -t734;
t865 = dq4.*t409.*-2.0;
t866 = -t737;
t867 = -t739;
t868 = -t741;
t871 = t475.*9.1e+1;
t872 = t478.*9.1e+1;
t873 = t481.*9.1e+1;
t874 = t483.*9.1e+1;
t875 = t487.*9.1e+1;
t876 = t490.*9.1e+1;
t878 = t486.*1.0e+2;
t881 = t491.*1.0e+2;
t882 = t493.*1.0e+2;
t883 = (dq1.*t139)./5.0e+1;
t884 = (dq1.*t149)./5.0e+1;
t885 = (dq4.*t141)./5.0e+1;
t886 = (dq5.*t142)./5.0e+1;
t888 = (dq5.*t156)./5.0e+1;
t889 = (dq4.*t169)./5.0e+1;
t892 = -t757;
t893 = -t760;
t894 = dq4.*t433.*-2.0;
t895 = -t762;
t896 = -t763;
t897 = t520.*9.1e+1;
t898 = t526.*9.1e+1;
t899 = t529.*9.1e+1;
t906 = (dq1.*t188)./5.0e+1;
t907 = (dq1.*t198)./5.0e+1;
t908 = (dq4.*t190)./5.0e+1;
t909 = (dq5.*t186)./5.0e+1;
t910 = (dq5.*t191)./5.0e+1;
t911 = t558.*9.1e+1;
t912 = t560.*9.1e+1;
t913 = t561.*9.1e+1;
t914 = (dq5.*t230)./5.0e+1;
t916 = -t784;
t934 = -t824;
t941 = -t839;
t943 = -t842;
t947 = t25.*t120.*1.82e+2;
t948 = dq5.*t6.*t121.*2.0e+2;
t949 = t25.*t132.*1.82e+2;
t951 = t25.*t151.*1.82e+2;
t952 = dq1.*t6.*t139.*2.0e+2;
t954 = dq1.*t6.*t149.*2.0e+2;
t955 = dq4.*t6.*t141.*2.0e+2;
t956 = dq6.*t11.*t114.*2.0e+2;
t957 = dq6.*t6.*t135.*2.0e+2;
t958 = dq5.*t6.*t142.*2.0e+2;
t959 = dq6.*t6.*t145.*2.0e+2;
C = ft_2({dq1,dq2,dq3,dq4,dq5,dq6,q3,t10,t100,t1008,t101,t1017,t102,t1020,t1021,t1025,t103,t1030,t1031,t1032,t1035,t1036,t1037,t1038,t104,t1040,t1041,t1043,t105,t1051,t1055,t1056,t1058,t1059,t106,t1064,t107,t108,t1082,t1084,t1085,t1086,t1087,t109,t11,t110,t1104,t1107,t1109,t111,t1110,t112,t1126,t113,t1137,t1148,t1149,t1152,t1158,t1167,t1168,t118,t1180,t12,t120,t1202,t1205,t1208,t1209,t121,t1210,t1211,t1213,t1217,t1218,t1219,t1220,t1221,t1222,t1223,t1224,t1225,t1226,t123,t1234,t1235,t1241,t1242,t1243,t1244,t1247,t1248,t1257,t1262,t1287,t1288,t129,t1290,t1291,t13,t130,t131,t1317,t132,t133,t134,t135,t136,t137,t1374,t138,t139,t1399,t140,t1405,t1407,t141,t142,t1420,t1422,t1425,t143,t144,t145,t146,t147,t148,t149,t150,t151,t1511,t152,t153,t154,t155,t156,t157,t158,t159,t16,t160,t161,t162,t163,t164,t166,t168,t169,t170,t171,t172,t173,t175,t176,t177,t178,t179,t18,t180,t181,t182,t183,t184,t185,t186,t187,t188,t189,t19,t190,t191,t192,t193,t194,t195,t196,t197,t198,t199,t2,t20,t200,t201,t202,t203,t204,t205,t206,t207,t208,t209,t21,t211,t212,t213,t214,t215,t216,t217,t218,t219,t22,t220,t221,t222,t223,t224,t225,t226,t227,t229,t23,t230,t231,t233,t235,t24,t240,t241,t242,t245,t246,t247,t249,t25,t250,t251,t252,t253,t254,t256,t257,t258,t259,t26,t260,t261,t262,t263,t264,t265,t266,t267,t268,t269,t271,t273,t274,t278,t279,t28,t284,t285,t286,t288,t29,t290,t291,t292,t294,t295,t296,t297,t298,t299,t3,t30,t300,t301,t302,t303,t304,t305,t306,t308,t31,t311,t312,t313,t314,t315,t316,t317,t318,t319,t32,t320,t321,t322,t323,t326,t328,t329,t33,t330,t331,t332,t333,t334,t336,t337,t338,t340,t341,t342,t343,t344,t345,t346,t348,t349,t35,t350,t351,t352,t353,t354,t355,t356,t357,t358,t359,t36,t360,t361,t362,t363,t364,t365,t366,t367,t368,t369,t370,t371,t372,t373,t374,t375,t376,t377,t378,t379,t38,t380,t381,t382,t383,t384,t385,t386,t387,t388,t389,t39,t391,t392,t393,t394,t395,t396,t397,t398,t399,t4,t40,t400,t401,t402,t403,t404,t405,t406,t407,t408,t409,t410,t411,t413,t414,t415,t417,t419,t421,t424,t425,t428,t429,t43,t430,t431,t432,t433,t434,t435,t437,t439,t44,t440,t441,t442,t443,t444,t445,t446,t447,t448,t449,t45,t450,t451,t452,t453,t454,t455,t456,t457,t458,t459,t460,t461,t463,t468,t469,t47,t470,t471,t473,t474,t475,t476,t477,t478,t479,t48,t480,t481,t482,t483,t485,t486,t487,t488,t49,t490,t491,t493,t494,t495,t496,t497,t498,t499,t5,t50,t500,t501,t502,t503,t504,t505,t507,t508,t509,t51,t510,t511,t512,t514,t515,t516,t517,t518,t519,t520,t522,t523,t524,t525,t526,t528,t529,t53,t531,t532,t533,t534,t535,t536,t537,t538,t539,t54,t540,t541,t542,t543,t544,t545,t546,t547,t548,t549,t55,t550,t551,t552,t553,t554,t555,t556,t557,t558,t559,t56,t560,t561,t562,t563,t564,t565,t567,t568,t569,t57,t570,t571,t572,t575,t577,t578,t579,t58,t580,t581,t582,t583,t584,t585,t586,t587,t588,t589,t59,t590,t591,t593,t595,t598,t599,t6,t60,t603,t604,t605,t608,t609,t61,t610,t611,t612,t615,t616,t617,t618,t619,t62,t623,t625,t626,t627,t628,t629,t63,t630,t631,t632,t633,t634,t635,t636,t638,t642,t643,t646,t649,t65,t651,t652,t653,t654,t655,t656,t657,t658,t659,t66,t660,t661,t662,t664,t666,t667,t668,t67,t672,t674,t675,t676,t677,t679,t680,t681,t682,t683,t684,t685,t686,t687,t688,t689,t69,t691,t692,t693,t694,t697,t698,t699,t7,t70,t700,t701,t702,t703,t704,t705,t706,t707,t708,t709,t71,t710,t711,t712,t713,t714,t715,t716,t717,t718,t719,t72,t721,t722,t723,t724,t725,t726,t727,t728,t729,t73,t730,t731,t732,t735,t738,t74,t740,t742,t743,t744,t745,t746,t747,t748,t749,t75,t750,t751,t752,t753,t754,t755,t756,t758,t759,t76,t764,t765,t766,t767,t768,t769,t77,t770,t771,t772,t773,t774,t775,t776,t777,t778,t779,t78,t780,t781,t782,t783,t785,t786,t79,t790,t791,t793,t794,t795,t796,t797,t798,t799,t8,t800,t801,t802,t803,t804,t805,t806,t807,t808,t809,t81,t810,t811,t812,t813,t814,t815,t816,t817,t818,t819,t82,t820,t821,t822,t823,t825,t826,t827,t828,t829,t83,t831,t832,t833,t834,t835,t836,t837,t838,t84,t840,t841,t843,t844,t845,t846,t847,t848,t849,t85,t850,t851,t856,t858,t859,t86,t860,t861,t863,t864,t865,t866,t867,t868,t87,t871,t872,t873,t874,t875,t876,t877,t878,t879,t88,t881,t882,t883,t884,t885,t886,t887,t888,t889,t89,t892,t893,t894,t895,t896,t897,t898,t899,t9,t900,t901,t902,t903,t904,t905,t906,t907,t908,t909,t910,t911,t912,t913,t914,t915,t916,t918,t919,t920,t921,t922,t923,t93,t934,t937,t94,t941,t943,t945,t947,t948,t949,t95,t950,t951,t952,t953,t954,t955,t956,t957,t958,t959,t96,t965,t966,t967,t97,t971,t98,t989,t99,t990,t991,t997});
end
function C = ft_2(ct)
dq1 = ct{1};
dq2 = ct{2};
dq3 = ct{3};
dq4 = ct{4};
dq5 = ct{5};
dq6 = ct{6};
q3 = ct{7};
t10 = ct{8};
t100 = ct{9};
t1008 = ct{10};
t101 = ct{11};
t1017 = ct{12};
t102 = ct{13};
t1020 = ct{14};
t1021 = ct{15};
t1025 = ct{16};
t103 = ct{17};
t1030 = ct{18};
t1031 = ct{19};
t1032 = ct{20};
t1035 = ct{21};
t1036 = ct{22};
t1037 = ct{23};
t1038 = ct{24};
t104 = ct{25};
t1040 = ct{26};
t1041 = ct{27};
t1043 = ct{28};
t105 = ct{29};
t1051 = ct{30};
t1055 = ct{31};
t1056 = ct{32};
t1058 = ct{33};
t1059 = ct{34};
t106 = ct{35};
t1064 = ct{36};
t107 = ct{37};
t108 = ct{38};
t1082 = ct{39};
t1084 = ct{40};
t1085 = ct{41};
t1086 = ct{42};
t1087 = ct{43};
t109 = ct{44};
t11 = ct{45};
t110 = ct{46};
t1104 = ct{47};
t1107 = ct{48};
t1109 = ct{49};
t111 = ct{50};
t1110 = ct{51};
t112 = ct{52};
t1126 = ct{53};
t113 = ct{54};
t1137 = ct{55};
t1148 = ct{56};
t1149 = ct{57};
t1152 = ct{58};
t1158 = ct{59};
t1167 = ct{60};
t1168 = ct{61};
t118 = ct{62};
t1180 = ct{63};
t12 = ct{64};
t120 = ct{65};
t1202 = ct{66};
t1205 = ct{67};
t1208 = ct{68};
t1209 = ct{69};
t121 = ct{70};
t1210 = ct{71};
t1211 = ct{72};
t1213 = ct{73};
t1217 = ct{74};
t1218 = ct{75};
t1219 = ct{76};
t1220 = ct{77};
t1221 = ct{78};
t1222 = ct{79};
t1223 = ct{80};
t1224 = ct{81};
t1225 = ct{82};
t1226 = ct{83};
t123 = ct{84};
t1234 = ct{85};
t1235 = ct{86};
t1241 = ct{87};
t1242 = ct{88};
t1243 = ct{89};
t1244 = ct{90};
t1247 = ct{91};
t1248 = ct{92};
t1257 = ct{93};
t1262 = ct{94};
t1287 = ct{95};
t1288 = ct{96};
t129 = ct{97};
t1290 = ct{98};
t1291 = ct{99};
t13 = ct{100};
t130 = ct{101};
t131 = ct{102};
t1317 = ct{103};
t132 = ct{104};
t133 = ct{105};
t134 = ct{106};
t135 = ct{107};
t136 = ct{108};
t137 = ct{109};
t1374 = ct{110};
t138 = ct{111};
t139 = ct{112};
t1399 = ct{113};
t140 = ct{114};
t1405 = ct{115};
t1407 = ct{116};
t141 = ct{117};
t142 = ct{118};
t1420 = ct{119};
t1422 = ct{120};
t1425 = ct{121};
t143 = ct{122};
t144 = ct{123};
t145 = ct{124};
t146 = ct{125};
t147 = ct{126};
t148 = ct{127};
t149 = ct{128};
t150 = ct{129};
t151 = ct{130};
t1511 = ct{131};
t152 = ct{132};
t153 = ct{133};
t154 = ct{134};
t155 = ct{135};
t156 = ct{136};
t157 = ct{137};
t158 = ct{138};
t159 = ct{139};
t16 = ct{140};
t160 = ct{141};
t161 = ct{142};
t162 = ct{143};
t163 = ct{144};
t164 = ct{145};
t166 = ct{146};
t168 = ct{147};
t169 = ct{148};
t170 = ct{149};
t171 = ct{150};
t172 = ct{151};
t173 = ct{152};
t175 = ct{153};
t176 = ct{154};
t177 = ct{155};
t178 = ct{156};
t179 = ct{157};
t18 = ct{158};
t180 = ct{159};
t181 = ct{160};
t182 = ct{161};
t183 = ct{162};
t184 = ct{163};
t185 = ct{164};
t186 = ct{165};
t187 = ct{166};
t188 = ct{167};
t189 = ct{168};
t19 = ct{169};
t190 = ct{170};
t191 = ct{171};
t192 = ct{172};
t193 = ct{173};
t194 = ct{174};
t195 = ct{175};
t196 = ct{176};
t197 = ct{177};
t198 = ct{178};
t199 = ct{179};
t2 = ct{180};
t20 = ct{181};
t200 = ct{182};
t201 = ct{183};
t202 = ct{184};
t203 = ct{185};
t204 = ct{186};
t205 = ct{187};
t206 = ct{188};
t207 = ct{189};
t208 = ct{190};
t209 = ct{191};
t21 = ct{192};
t211 = ct{193};
t212 = ct{194};
t213 = ct{195};
t214 = ct{196};
t215 = ct{197};
t216 = ct{198};
t217 = ct{199};
t218 = ct{200};
t219 = ct{201};
t22 = ct{202};
t220 = ct{203};
t221 = ct{204};
t222 = ct{205};
t223 = ct{206};
t224 = ct{207};
t225 = ct{208};
t226 = ct{209};
t227 = ct{210};
t229 = ct{211};
t23 = ct{212};
t230 = ct{213};
t231 = ct{214};
t233 = ct{215};
t235 = ct{216};
t24 = ct{217};
t240 = ct{218};
t241 = ct{219};
t242 = ct{220};
t245 = ct{221};
t246 = ct{222};
t247 = ct{223};
t249 = ct{224};
t25 = ct{225};
t250 = ct{226};
t251 = ct{227};
t252 = ct{228};
t253 = ct{229};
t254 = ct{230};
t256 = ct{231};
t257 = ct{232};
t258 = ct{233};
t259 = ct{234};
t26 = ct{235};
t260 = ct{236};
t261 = ct{237};
t262 = ct{238};
t263 = ct{239};
t264 = ct{240};
t265 = ct{241};
t266 = ct{242};
t267 = ct{243};
t268 = ct{244};
t269 = ct{245};
t271 = ct{246};
t273 = ct{247};
t274 = ct{248};
t278 = ct{249};
t279 = ct{250};
t28 = ct{251};
t284 = ct{252};
t285 = ct{253};
t286 = ct{254};
t288 = ct{255};
t29 = ct{256};
t290 = ct{257};
t291 = ct{258};
t292 = ct{259};
t294 = ct{260};
t295 = ct{261};
t296 = ct{262};
t297 = ct{263};
t298 = ct{264};
t299 = ct{265};
t3 = ct{266};
t30 = ct{267};
t300 = ct{268};
t301 = ct{269};
t302 = ct{270};
t303 = ct{271};
t304 = ct{272};
t305 = ct{273};
t306 = ct{274};
t308 = ct{275};
t31 = ct{276};
t311 = ct{277};
t312 = ct{278};
t313 = ct{279};
t314 = ct{280};
t315 = ct{281};
t316 = ct{282};
t317 = ct{283};
t318 = ct{284};
t319 = ct{285};
t32 = ct{286};
t320 = ct{287};
t321 = ct{288};
t322 = ct{289};
t323 = ct{290};
t326 = ct{291};
t328 = ct{292};
t329 = ct{293};
t33 = ct{294};
t330 = ct{295};
t331 = ct{296};
t332 = ct{297};
t333 = ct{298};
t334 = ct{299};
t336 = ct{300};
t337 = ct{301};
t338 = ct{302};
t340 = ct{303};
t341 = ct{304};
t342 = ct{305};
t343 = ct{306};
t344 = ct{307};
t345 = ct{308};
t346 = ct{309};
t348 = ct{310};
t349 = ct{311};
t35 = ct{312};
t350 = ct{313};
t351 = ct{314};
t352 = ct{315};
t353 = ct{316};
t354 = ct{317};
t355 = ct{318};
t356 = ct{319};
t357 = ct{320};
t358 = ct{321};
t359 = ct{322};
t36 = ct{323};
t360 = ct{324};
t361 = ct{325};
t362 = ct{326};
t363 = ct{327};
t364 = ct{328};
t365 = ct{329};
t366 = ct{330};
t367 = ct{331};
t368 = ct{332};
t369 = ct{333};
t370 = ct{334};
t371 = ct{335};
t372 = ct{336};
t373 = ct{337};
t374 = ct{338};
t375 = ct{339};
t376 = ct{340};
t377 = ct{341};
t378 = ct{342};
t379 = ct{343};
t38 = ct{344};
t380 = ct{345};
t381 = ct{346};
t382 = ct{347};
t383 = ct{348};
t384 = ct{349};
t385 = ct{350};
t386 = ct{351};
t387 = ct{352};
t388 = ct{353};
t389 = ct{354};
t39 = ct{355};
t391 = ct{356};
t392 = ct{357};
t393 = ct{358};
t394 = ct{359};
t395 = ct{360};
t396 = ct{361};
t397 = ct{362};
t398 = ct{363};
t399 = ct{364};
t4 = ct{365};
t40 = ct{366};
t400 = ct{367};
t401 = ct{368};
t402 = ct{369};
t403 = ct{370};
t404 = ct{371};
t405 = ct{372};
t406 = ct{373};
t407 = ct{374};
t408 = ct{375};
t409 = ct{376};
t410 = ct{377};
t411 = ct{378};
t413 = ct{379};
t414 = ct{380};
t415 = ct{381};
t417 = ct{382};
t419 = ct{383};
t421 = ct{384};
t424 = ct{385};
t425 = ct{386};
t428 = ct{387};
t429 = ct{388};
t43 = ct{389};
t430 = ct{390};
t431 = ct{391};
t432 = ct{392};
t433 = ct{393};
t434 = ct{394};
t435 = ct{395};
t437 = ct{396};
t439 = ct{397};
t44 = ct{398};
t440 = ct{399};
t441 = ct{400};
t442 = ct{401};
t443 = ct{402};
t444 = ct{403};
t445 = ct{404};
t446 = ct{405};
t447 = ct{406};
t448 = ct{407};
t449 = ct{408};
t45 = ct{409};
t450 = ct{410};
t451 = ct{411};
t452 = ct{412};
t453 = ct{413};
t454 = ct{414};
t455 = ct{415};
t456 = ct{416};
t457 = ct{417};
t458 = ct{418};
t459 = ct{419};
t460 = ct{420};
t461 = ct{421};
t463 = ct{422};
t468 = ct{423};
t469 = ct{424};
t47 = ct{425};
t470 = ct{426};
t471 = ct{427};
t473 = ct{428};
t474 = ct{429};
t475 = ct{430};
t476 = ct{431};
t477 = ct{432};
t478 = ct{433};
t479 = ct{434};
t48 = ct{435};
t480 = ct{436};
t481 = ct{437};
t482 = ct{438};
t483 = ct{439};
t485 = ct{440};
t486 = ct{441};
t487 = ct{442};
t488 = ct{443};
t49 = ct{444};
t490 = ct{445};
t491 = ct{446};
t493 = ct{447};
t494 = ct{448};
t495 = ct{449};
t496 = ct{450};
t497 = ct{451};
t498 = ct{452};
t499 = ct{453};
t5 = ct{454};
t50 = ct{455};
t500 = ct{456};
t501 = ct{457};
t502 = ct{458};
t503 = ct{459};
t504 = ct{460};
t505 = ct{461};
t507 = ct{462};
t508 = ct{463};
t509 = ct{464};
t51 = ct{465};
t510 = ct{466};
t511 = ct{467};
t512 = ct{468};
t514 = ct{469};
t515 = ct{470};
t516 = ct{471};
t517 = ct{472};
t518 = ct{473};
t519 = ct{474};
t520 = ct{475};
t522 = ct{476};
t523 = ct{477};
t524 = ct{478};
t525 = ct{479};
t526 = ct{480};
t528 = ct{481};
t529 = ct{482};
t53 = ct{483};
t531 = ct{484};
t532 = ct{485};
t533 = ct{486};
t534 = ct{487};
t535 = ct{488};
t536 = ct{489};
t537 = ct{490};
t538 = ct{491};
t539 = ct{492};
t54 = ct{493};
t540 = ct{494};
t541 = ct{495};
t542 = ct{496};
t543 = ct{497};
t544 = ct{498};
t545 = ct{499};
t546 = ct{500};
t547 = ct{501};
t548 = ct{502};
t549 = ct{503};
t55 = ct{504};
t550 = ct{505};
t551 = ct{506};
t552 = ct{507};
t553 = ct{508};
t554 = ct{509};
t555 = ct{510};
t556 = ct{511};
t557 = ct{512};
t558 = ct{513};
t559 = ct{514};
t56 = ct{515};
t560 = ct{516};
t561 = ct{517};
t562 = ct{518};
t563 = ct{519};
t564 = ct{520};
t565 = ct{521};
t567 = ct{522};
t568 = ct{523};
t569 = ct{524};
t57 = ct{525};
t570 = ct{526};
t571 = ct{527};
t572 = ct{528};
t575 = ct{529};
t577 = ct{530};
t578 = ct{531};
t579 = ct{532};
t58 = ct{533};
t580 = ct{534};
t581 = ct{535};
t582 = ct{536};
t583 = ct{537};
t584 = ct{538};
t585 = ct{539};
t586 = ct{540};
t587 = ct{541};
t588 = ct{542};
t589 = ct{543};
t59 = ct{544};
t590 = ct{545};
t591 = ct{546};
t593 = ct{547};
t595 = ct{548};
t598 = ct{549};
t599 = ct{550};
t6 = ct{551};
t60 = ct{552};
t603 = ct{553};
t604 = ct{554};
t605 = ct{555};
t608 = ct{556};
t609 = ct{557};
t61 = ct{558};
t610 = ct{559};
t611 = ct{560};
t612 = ct{561};
t615 = ct{562};
t616 = ct{563};
t617 = ct{564};
t618 = ct{565};
t619 = ct{566};
t62 = ct{567};
t623 = ct{568};
t625 = ct{569};
t626 = ct{570};
t627 = ct{571};
t628 = ct{572};
t629 = ct{573};
t63 = ct{574};
t630 = ct{575};
t631 = ct{576};
t632 = ct{577};
t633 = ct{578};
t634 = ct{579};
t635 = ct{580};
t636 = ct{581};
t638 = ct{582};
t642 = ct{583};
t643 = ct{584};
t646 = ct{585};
t649 = ct{586};
t65 = ct{587};
t651 = ct{588};
t652 = ct{589};
t653 = ct{590};
t654 = ct{591};
t655 = ct{592};
t656 = ct{593};
t657 = ct{594};
t658 = ct{595};
t659 = ct{596};
t66 = ct{597};
t660 = ct{598};
t661 = ct{599};
t662 = ct{600};
t664 = ct{601};
t666 = ct{602};
t667 = ct{603};
t668 = ct{604};
t67 = ct{605};
t672 = ct{606};
t674 = ct{607};
t675 = ct{608};
t676 = ct{609};
t677 = ct{610};
t679 = ct{611};
t680 = ct{612};
t681 = ct{613};
t682 = ct{614};
t683 = ct{615};
t684 = ct{616};
t685 = ct{617};
t686 = ct{618};
t687 = ct{619};
t688 = ct{620};
t689 = ct{621};
t69 = ct{622};
t691 = ct{623};
t692 = ct{624};
t693 = ct{625};
t694 = ct{626};
t697 = ct{627};
t698 = ct{628};
t699 = ct{629};
t7 = ct{630};
t70 = ct{631};
t700 = ct{632};
t701 = ct{633};
t702 = ct{634};
t703 = ct{635};
t704 = ct{636};
t705 = ct{637};
t706 = ct{638};
t707 = ct{639};
t708 = ct{640};
t709 = ct{641};
t71 = ct{642};
t710 = ct{643};
t711 = ct{644};
t712 = ct{645};
t713 = ct{646};
t714 = ct{647};
t715 = ct{648};
t716 = ct{649};
t717 = ct{650};
t718 = ct{651};
t719 = ct{652};
t72 = ct{653};
t721 = ct{654};
t722 = ct{655};
t723 = ct{656};
t724 = ct{657};
t725 = ct{658};
t726 = ct{659};
t727 = ct{660};
t728 = ct{661};
t729 = ct{662};
t73 = ct{663};
t730 = ct{664};
t731 = ct{665};
t732 = ct{666};
t735 = ct{667};
t738 = ct{668};
t74 = ct{669};
t740 = ct{670};
t742 = ct{671};
t743 = ct{672};
t744 = ct{673};
t745 = ct{674};
t746 = ct{675};
t747 = ct{676};
t748 = ct{677};
t749 = ct{678};
t75 = ct{679};
t750 = ct{680};
t751 = ct{681};
t752 = ct{682};
t753 = ct{683};
t754 = ct{684};
t755 = ct{685};
t756 = ct{686};
t758 = ct{687};
t759 = ct{688};
t76 = ct{689};
t764 = ct{690};
t765 = ct{691};
t766 = ct{692};
t767 = ct{693};
t768 = ct{694};
t769 = ct{695};
t77 = ct{696};
t770 = ct{697};
t771 = ct{698};
t772 = ct{699};
t773 = ct{700};
t774 = ct{701};
t775 = ct{702};
t776 = ct{703};
t777 = ct{704};
t778 = ct{705};
t779 = ct{706};
t78 = ct{707};
t780 = ct{708};
t781 = ct{709};
t782 = ct{710};
t783 = ct{711};
t785 = ct{712};
t786 = ct{713};
t79 = ct{714};
t790 = ct{715};
t791 = ct{716};
t793 = ct{717};
t794 = ct{718};
t795 = ct{719};
t796 = ct{720};
t797 = ct{721};
t798 = ct{722};
t799 = ct{723};
t8 = ct{724};
t800 = ct{725};
t801 = ct{726};
t802 = ct{727};
t803 = ct{728};
t804 = ct{729};
t805 = ct{730};
t806 = ct{731};
t807 = ct{732};
t808 = ct{733};
t809 = ct{734};
t81 = ct{735};
t810 = ct{736};
t811 = ct{737};
t812 = ct{738};
t813 = ct{739};
t814 = ct{740};
t815 = ct{741};
t816 = ct{742};
t817 = ct{743};
t818 = ct{744};
t819 = ct{745};
t82 = ct{746};
t820 = ct{747};
t821 = ct{748};
t822 = ct{749};
t823 = ct{750};
t825 = ct{751};
t826 = ct{752};
t827 = ct{753};
t828 = ct{754};
t829 = ct{755};
t83 = ct{756};
t831 = ct{757};
t832 = ct{758};
t833 = ct{759};
t834 = ct{760};
t835 = ct{761};
t836 = ct{762};
t837 = ct{763};
t838 = ct{764};
t84 = ct{765};
t840 = ct{766};
t841 = ct{767};
t843 = ct{768};
t844 = ct{769};
t845 = ct{770};
t846 = ct{771};
t847 = ct{772};
t848 = ct{773};
t849 = ct{774};
t85 = ct{775};
t850 = ct{776};
t851 = ct{777};
t856 = ct{778};
t858 = ct{779};
t859 = ct{780};
t86 = ct{781};
t860 = ct{782};
t861 = ct{783};
t863 = ct{784};
t864 = ct{785};
t865 = ct{786};
t866 = ct{787};
t867 = ct{788};
t868 = ct{789};
t87 = ct{790};
t871 = ct{791};
t872 = ct{792};
t873 = ct{793};
t874 = ct{794};
t875 = ct{795};
t876 = ct{796};
t877 = ct{797};
t878 = ct{798};
t879 = ct{799};
t88 = ct{800};
t881 = ct{801};
t882 = ct{802};
t883 = ct{803};
t884 = ct{804};
t885 = ct{805};
t886 = ct{806};
t887 = ct{807};
t888 = ct{808};
t889 = ct{809};
t89 = ct{810};
t892 = ct{811};
t893 = ct{812};
t894 = ct{813};
t895 = ct{814};
t896 = ct{815};
t897 = ct{816};
t898 = ct{817};
t899 = ct{818};
t9 = ct{819};
t900 = ct{820};
t901 = ct{821};
t902 = ct{822};
t903 = ct{823};
t904 = ct{824};
t905 = ct{825};
t906 = ct{826};
t907 = ct{827};
t908 = ct{828};
t909 = ct{829};
t910 = ct{830};
t911 = ct{831};
t912 = ct{832};
t913 = ct{833};
t914 = ct{834};
t915 = ct{835};
t916 = ct{836};
t918 = ct{837};
t919 = ct{838};
t920 = ct{839};
t921 = ct{840};
t922 = ct{841};
t923 = ct{842};
t93 = ct{843};
t934 = ct{844};
t937 = ct{845};
t94 = ct{846};
t941 = ct{847};
t943 = ct{848};
t945 = ct{849};
t947 = ct{850};
t948 = ct{851};
t949 = ct{852};
t95 = ct{853};
t950 = ct{854};
t951 = ct{855};
t952 = ct{856};
t953 = ct{857};
t954 = ct{858};
t955 = ct{859};
t956 = ct{860};
t957 = ct{861};
t958 = ct{862};
t959 = ct{863};
t96 = ct{864};
t965 = ct{865};
t966 = ct{866};
t967 = ct{867};
t97 = ct{868};
t971 = ct{869};
t98 = ct{870};
t989 = ct{871};
t99 = ct{872};
t990 = ct{873};
t991 = ct{874};
t997 = ct{875};
t960 = t25.*t172.*2.0e+2;
t961 = dq5.*t6.*t156.*2.0e+2;
t964 = t25.*t181.*1.82e+2;
t969 = dq1.*t7.*t159.*2.0e+2;
t970 = dq4.*t11.*t130.*2.0e+2;
t972 = dq1.*t7.*t171.*2.0e+2;
t973 = dq6.*t6.*t177.*2.0e+2;
t974 = dq4.*t6.*t190.*2.0e+2;
t975 = dq6.*t11.*t134.*2.0e+2;
t976 = dq5.*t6.*t186.*2.0e+2;
t977 = dq6.*t7.*t152.*2.0e+2;
t978 = dq5.*t6.*t191.*2.0e+2;
t979 = dq6.*t11.*t139.*2.0e+2;
t980 = dq6.*t6.*t194.*2.0e+2;
t981 = dq6.*t11.*t149.*2.0e+2;
t982 = dq6.*t11.*t154.*2.0e+2;
t983 = dq6.*t11.*t163.*2.0e+2;
t988 = dq4.*t407.*1.82e+2;
t992 = dq4.*t11.*t179.*2.0e+2;
t993 = dq6.*t6.*t227.*2.0e+2;
t994 = dq5.*t6.*t230.*2.0e+2;
t995 = dq6.*t11.*t188.*2.0e+2;
t996 = dq6.*t11.*t189.*2.0e+2;
t998 = t25.*t241.*2.0e+2;
t999 = dq6.*t11.*t198.*2.0e+2;
t1000 = dq6.*t11.*t204.*2.0e+2;
t1001 = dq6.*t425.*2.0e+2;
t1002 = dq6.*t11.*t212.*2.0e+2;
t1006 = -t877;
t1007 = -t879;
t1011 = dq4.*t433.*1.82e+2;
t1012 = dq6.*t11.*t231.*2.0e+2;
t1016 = -t915;
t1018 = t6.*t364.*1.0e+2;
t1019 = t32.*t172.*1.0e+2;
t1022 = t28.*t241.*1.0e+2;
t1023 = t334./1.0e+2;
t1024 = t343./1.0e+2;
t1026 = t32.*t241.*1.0e+2;
t1027 = t356./1.0e+2;
t1028 = t364./1.0e+2;
t1029 = t377./1.0e+2;
t1033 = t408./1.0e+2;
t1034 = t415./1.0e+2;
t1039 = t435./1.0e+2;
t1042 = t45+t246;
t1044 = t29+t322;
t1045 = t36+t303;
t1046 = t28+t278;
t1047 = t35+t313;
t1048 = t6.*t460.*1.0e+2;
t1049 = t6.*t461.*1.0e+2;
t1050 = t6.*t463.*1.0e+2;
t1052 = (t25.*t120)./5.0e+1;
t1063 = (t25.*t132)./5.0e+1;
t1065 = (t25.*t151)./5.0e+1;
t1067 = -t950;
t1070 = -t953;
t1075 = t698.*9.1e+1;
t1076 = t700.*9.1e+1;
t1077 = t702.*9.1e+1;
t1078 = t704.*9.1e+1;
t1079 = t6.*t520.*1.0e+2;
t1080 = t6.*t526.*1.0e+2;
t1081 = t6.*t529.*1.0e+2;
t1083 = (t25.*t181)./5.0e+1;
t1089 = -t971;
t1093 = t460./1.0e+2;
t1094 = t461./1.0e+2;
t1095 = t463./1.0e+2;
t1096 = t728.*9.1e+1;
t1097 = t729.*9.1e+1;
t1098 = t730.*9.1e+1;
t1099 = t731.*9.1e+1;
t1100 = t11.*t514.*1.0e+2;
t1101 = t11.*t517.*1.0e+2;
t1102 = t6.*t558.*1.0e+2;
t1103 = t11.*t522.*1.0e+2;
t1105 = t6.*t560.*1.0e+2;
t1106 = t6.*t561.*1.0e+2;
t1108 = (dq4.*t407)./5.0e+1;
t1112 = -t997;
t1117 = t475./1.0e+2;
t1118 = t478./1.0e+2;
t1119 = t481./1.0e+2;
t1120 = t483./1.0e+2;
t1121 = t487./1.0e+2;
t1122 = t490./1.0e+2;
t1123 = t11.*t556.*1.0e+2;
t1124 = t11.*t557.*1.0e+2;
t1125 = t11.*t559.*1.0e+2;
t1127 = (dq4.*t433)./5.0e+1;
t1130 = t520./1.0e+2;
t1131 = t526./1.0e+2;
t1132 = t529./1.0e+2;
t1133 = t558./1.0e+2;
t1134 = t560./1.0e+2;
t1135 = t561./1.0e+2;
t1136 = t850.^2;
t1138 = t6.*t334.*1.0e+2;
t1139 = t28.*t172.*1.0e+2;
t1140 = -t1020;
t1141 = -t1021;
t1143 = -t1025;
t1150 = t6.*t25.*t120.*2.0e+2;
t1153 = t6.*t25.*t132.*2.0e+2;
t1154 = t39.*t172.*2.0e+2;
t1155 = t6.*t25.*t151.*2.0e+2;
t1156 = t6.*t25.*t181.*2.0e+2;
t1157 = t50.*t172.*2.0e+2;
t1159 = dq6.*t11.*t334.*2.0e+2;
t1160 = t57.*t172.*2.0e+2;
t1161 = dq6.*t28.*t218.*2.0e+2;
t1165 = -t1051;
t1169 = t39.*t241.*2.0e+2;
t1170 = dq6.*t11.*t364.*2.0e+2;
t1171 = t67.*t172.*2.0e+2;
t1172 = dq6.*t32.*t218.*2.0e+2;
t1173 = -t1055;
t1174 = -t1056;
t1175 = -t1058;
t1176 = -t1059;
t1178 = -t1064;
t1181 = t50.*t241.*2.0e+2;
t1182 = t57.*t241.*2.0e+2;
t1183 = t67.*t241.*2.0e+2;
t1190 = -t1107;
t1191 = t6.*t849;
t1192 = t6.*t850;
t1196 = t11.*t849;
t1197 = t11.*t850;
t1227 = -t1180;
t1230 = t698./1.0e+2;
t1231 = t700./1.0e+2;
t1232 = t702./1.0e+2;
t1233 = t704./1.0e+2;
t1237 = t728./1.0e+2;
t1238 = t729./1.0e+2;
t1239 = t730./1.0e+2;
t1240 = t731./1.0e+2;
t1249 = t3.*t9.*t836;
t1261 = -t1244;
t1266 = t100+t604;
t1271 = t78+t629;
t1272 = t93+t619;
t1273 = t72+t610;
t1275 = t88+t632;
t1278 = -t1257;
t1279 = t45.*t836;
t1280 = t65.*t836;
t1281 = t6.*t1205;
t1282 = t11.*t1205;
t1283 = t6.*t1210;
t1284 = t11.*t1210;
t1285 = t6.*t1211;
t1286 = t11.*t1211;
t1302 = t246.*t836;
t1303 = t82+t83+t112;
t1316 = t96+t107+t290;
t1319 = t131+t136+t144;
t1321 = t258+t262+t268;
t1322 = t85+t286+t321;
t1323 = t73+t77+t617;
t1324 = t74+t300+t304;
t1325 = t109+t298+t315;
t1326 = t103+t306+t314;
t1329 = t1317.^2;
t1335 = t160+t169+t450;
t1337 = dq6.*t6.*t1317;
t1338 = dq6.*t11.*t1317;
t1371 = t55+t62+t148+t161+t168;
t1372 = t50+t57+t177+t184+t194;
t1375 = t56+t61+t147+t170+t453;
t1376 = t51+t1030+t1213;
t1383 = t66+t209+t216+t226+t398;
t1418 = -t1407;
t1424 = t82.*1.0e-1;
t1426 = t97.*1.0e-1;
t1463 = t274+t301+t1241+t1242+t1243;
t1513 = t1399+t1420;
t600 = -t468;
t601 = -t470;
t602 = -t471;
t606 = -t496;
t607 = -t500;
t613 = -t545;
t614 = -t550;
t620 = -t562;
t621 = -t563;
t622 = -t565;
t624 = -t568;
t637 = -t326;
t639 = -t328;
t640 = -t329;
t641 = -t333;
t644 = -t340;
t645 = -t341;
t647 = -t383;
t648 = -t387;
t650 = -t575;
t663 = -t428;
t665 = -t434;
t669 = -t585;
t670 = -t587;
t671 = -t588;
t673 = -t593;
t678 = dq6.*t328.*2.0;
t695 = dq4.*t352.*2.0;
t696 = dq6.*t350.*2.0;
t720 = dq4.*t387.*2.0;
t852 = -t676;
t853 = -t677;
t855 = -t688;
t857 = -t693;
t862 = -t732;
t869 = -t742;
t870 = -t743;
t890 = -t750;
t891 = -t751;
t917 = -t786;
t924 = -t794;
t925 = -t808;
t926 = -t812;
t927 = -t814;
t930 = -t815;
t931 = -t817;
t932 = -t818;
t933 = -t821;
t938 = -t831;
t939 = -t832;
t940 = -t838;
t942 = -t841;
t944 = -t843;
t946 = -t848;
t962 = dq4.*t352.*2.0e+2;
t963 = dq6.*t350.*2.0e+2;
t984 = -t858;
t985 = -t859;
t986 = -t860;
t987 = -t861;
t1003 = -t871;
t1004 = -t872;
t1005 = -t874;
t1009 = -t883;
t1010 = -t884;
t1013 = -t911;
t1014 = -t912;
t1015 = -t913;
t1053 = -t947;
t1054 = -t948;
t1057 = t684.*1.0e+2;
t1060 = t685.*1.0e+2;
t1061 = t686.*1.0e+2;
t1062 = t687.*1.0e+2;
t1066 = -t949;
t1068 = -t951;
t1069 = -t952;
t1071 = -t954;
t1072 = -t956;
t1073 = -t957;
t1074 = -t959;
t1088 = -t970;
t1090 = -t973;
t1091 = -t977;
t1092 = -t980;
t1111 = -t996;
t1113 = -t998;
t1114 = -t1000;
t1115 = -t1001;
t1116 = -t1002;
t1128 = -t1011;
t1129 = -t1012;
t1142 = -t1022;
t1144 = -t1026;
t1146 = -t1033;
t1147 = -t1034;
t1151 = -t1039;
t1162 = -t1048;
t1163 = -t1049;
t1164 = -t1050;
t1166 = -t1052;
t1177 = -t1063;
t1179 = -t1065;
t1184 = -t1093;
t1185 = -t1094;
t1186 = -t1095;
t1187 = -t1102;
t1188 = -t1105;
t1189 = -t1106;
t1193 = -t1117;
t1194 = -t1118;
t1195 = -t1120;
t1198 = -t1127;
t1199 = -t1133;
t1200 = -t1134;
t1201 = -t1135;
t1203 = dq6.*t1191;
t1204 = dq6.*t1192;
t1206 = dq6.*t1196;
t1207 = dq6.*t1197;
t1212 = -t1150;
t1214 = -t1153;
t1215 = -t1154;
t1216 = -t1155;
t1228 = -t1181;
t1229 = -t1182;
t1236 = -t1183;
t1245 = t1045.^2;
t1246 = t1046.^2;
t1252 = t6.*t1046;
t1253 = t6.*t1047;
t1254 = -t1191;
t1258 = t11.*t1046;
t1259 = t11.*t1047;
t1260 = -t1197;
t1267 = t110+t605;
t1274 = t75+t612;
t1276 = t16.*t1192;
t1277 = t16.*t1197;
t1296 = dq6.*t1281;
t1297 = dq6.*t1282;
t1298 = dq6.*t1283;
t1299 = dq6.*t1284;
t1300 = dq6.*t1285;
t1301 = dq6.*t1286;
t1304 = t30+t76+t317;
t1305 = t6.*t1275;
t1306 = t1249./1.0e+1;
t1307 = t11.*t1275;
t1310 = t1279./1.0e+1;
t1315 = t1280./1.0e+1;
t1327 = t95+t108+t630;
t1328 = t1316.^2;
t1330 = t250+t252+t320;
t1331 = t185+t193+t392;
t1332 = t178+t183+t397;
t1333 = t196+t215+t401;
t1334 = t129+t146+t446;
t1336 = t1322.^2;
t1339 = t846.*t1042;
t1340 = t6.*t1323;
t1341 = t6.*t1326;
t1342 = t11.*t1323;
t1343 = t11.*t1326;
t1344 = t296+t1281;
t1346 = t308+t1283;
t1347 = dq6.*t6.*t1322;
t1351 = dq6.*t11.*t1322;
t1355 = -t1338;
t1362 = t611+t1282;
t1363 = t618+t1284;
t1373 = t49+t58+t179+t192+t394;
t1379 = t846.*t1321;
t1380 = t6.*t1372;
t1381 = t11.*t1372;
t1382 = t69+t195+t208+t225+t404;
t1384 = t39+t135+t145+t247+t444;
t1385 = t44+t130+t137+t245+t449;
t1391 = t3.*t9.*t1371;
t1396 = t45.*t1371;
t1397 = t65.*t1371;
t1414 = t3.*t9.*t1383;
t1430 = -t1426;
t1437 = t1045.*t1375;
t1444 = t1326.*t1372;
t1445 = t1325.*t1371;
t1448 = t138+t150+t332+t336+t338+t342+t445;
t1449 = t158+t172+t346+t349+t351+t354+t456;
t1450 = t180+t187+t199+t366+t371+t376+t635;
t1452 = t143+t155+t162+t357+t365+t372+t667;
t1453 = t190+t203+t402+t407+t411+t417+t421;
t1457 = t1325.*t1383;
t1460 = t182+t197+t358+t363+t368+t395+t638;
t1461 = t264+t265+t1234+t1235+t1261;
t1464 = t141+t164+t362+t369+t375+t452+t664;
t1471 = t205+t211+t396+t409+t419+t642+t643;
t1472 = t201+t213+t348+t352+t405+t659+t662;
t1473 = t133+t140+t330+t344+t451+t653+t655;
t1495 = t26+t591+t697+t816+t941+t943+t945;
t1501 = t259+t263+t269+t481+t487+t490+t507+t511+t623;
t1502 = t256+t260+t267+t515+t518+t523+t538+t540+t598;
t1503 = t257+t261+t266+t514+t517+t522+t535+t539+t599;
t1512 = t271+t273+t302+t547+t549+t553+t724+t726+t727;
t1514 = t249+t251+t319+t494+t497+t499+t776+t777+t779;
t1520 = t142+t156+t181+t186+t359+t370+t374+t399+t454+t636;
t1522 = t154+t163+t188+t198+t356+t364+t377+t393+t448+t666;
t1532 = t157+t176+t202+t220+t350+t355+t403+t455+t658+t660;
t1534 = t207+t217+t240+t378+t388+t391+t406+t429+t431+t668;
t1542 = t121+t132+t151+t331+t337+t440+t442+t447+t656+t657;
t1543 = t134+t139+t149+t334+t343+t439+t441+t443+t652+t654;
t1637 = t1418+t1424+t1425;
t1647 = t111+t631+t887+t889+t918+t919+t1016+t1119+t1121+t1122+t1202;
t854 = -t678;
t1263 = dq6.*t1252;
t1264 = dq6.*t1253;
t1265 = -t1203;
t1268 = dq6.*t1258;
t1269 = dq6.*t1259;
t1270 = -t1206;
t1289 = -t1253;
t1292 = -t1258;
t1294 = t16.*t1252;
t1295 = t16.*t1258;
t1311 = -t1299;
t1312 = dq6.*t1305;
t1313 = dq6.*t1307;
t1314 = -t1301;
t1318 = -t1315;
t1345 = t6.*t1332;
t1348 = t6.*t1334;
t1349 = t11.*t1332;
t1350 = dq6.*t1340;
t1352 = t11.*t1334;
t1353 = dq6.*t1341;
t1354 = dq6.*t1342;
t1356 = dq6.*t1343;
t1357 = t3.*t9.*t1330;
t1358 = t16.*t1340;
t1359 = t16.*t1341;
t1360 = t16.*t1342;
t1361 = t16.*t1343;
t1364 = -t1347;
t1377 = t1259+t1285;
t1378 = t1196+t1305;
t1387 = t1254+t1307;
t1388 = -t1379;
t1389 = dq6.*t1380.*2.0;
t1390 = dq6.*t1381.*2.0;
t1392 = t6.*t1373;
t1393 = t11.*t1373;
t1400 = t6.*t1384;
t1401 = t6.*t1385;
t1403 = t11.*t1384;
t1404 = t11.*t1385;
t1406 = -t1396;
t1410 = t1391./1.0e+1;
t1411 = t1192+t1342;
t1413 = t3.*t9.*t1382;
t1421 = t1396./1.0e+1;
t1423 = t1397./1.0e+1;
t1427 = t1260+t1340;
t1428 = t1252+t1343;
t1432 = t1414./1.0e+1;
t1434 = (t1197-t1340).^2;
t1435 = (t1258-t1341).^2;
t1436 = t850.*t1373;
t1438 = t1042.*t1382;
t1439 = t1045.*t1382;
t1441 = t1046.*t1385;
t1446 = -t1445;
t1447 = t1323.*t1373;
t1451 = t206+t218+t223+t379+t384+t386+t640;
t1454 = t1445./1.0e+1;
t1456 = t1325.*t1382;
t1458 = t1323.*t1384;
t1459 = t1326.*t1385;
t1462 = t1339.*1.0e-1;
t1466 = t6.*t1453;
t1467 = t11.*t1453;
t1468 = -t1457;
t1474 = t153+t166+t173+t437+t647+t648+t649;
t1475 = t6.*t1460;
t1476 = t11.*t1460;
t1477 = t6.*t1464;
t1478 = t11.*t1464;
t1480 = t1457./1.0e+1;
t1483 = t6.*t1473;
t1484 = t11.*t1473;
t1485 = t1371.*t1382;
t1486 = t1372.*t1385;
t1487 = t1379.*1.0e-1;
t1489 = t1373.*t1384;
t1491 = t850.*t1448;
t1492 = t1046.*t1450;
t1493 = t1046.*t1452;
t1496 = t1045.*t1449;
t1498 = t850.*t1471;
t1506 = t1045.*t1472;
t1508 = t6.*t1503;
t1509 = t11.*t1503;
t1510 = t254+t473+t476+t480+t495+t498+t571+t572+t621;
t1516 = t1317.*t1453;
t1517 = t159+t171+t175+t200+t214+t221+t345+t353+t661+t663;
t1521 = t1437.*1.0e-1;
t1523 = t6.*t1514;
t1524 = t11.*t1514;
t1525 = t1322.*t1460;
t1527 = t1317.*t1473;
t1528 = t1322.*t1464;
t1531 = t219+t222+t235+t380+t385+t389+t400+t430+t432+t639;
t1533 = t3.*t9.*t1512;
t1537 = t6.*t1520;
t1538 = t11.*t1520;
t1539 = t6.*t1522;
t1540 = t11.*t1522;
t1549 = t1045.*t1501;
t1550 = t1046.*t1502;
t1551 = t6.*t1542;
t1552 = t6.*t1543;
t1553 = t11.*t1542;
C = ft_3({dq1,dq2,dq3,dq4,dq5,dq6,q3,t10,t1003,t1004,t1005,t1006,t1007,t1008,t1009,t101,t1010,t1013,t1014,t1015,t1017,t1018,t1019,t102,t1023,t1024,t1027,t1028,t1029,t103,t1030,t1031,t1032,t1035,t1036,t1037,t1038,t104,t1040,t1041,t1042,t1043,t1044,t1045,t1046,t1047,t105,t1053,t1054,t1057,t106,t1060,t1061,t1062,t1066,t1067,t1068,t1069,t1070,t1071,t1072,t1073,t1074,t1075,t1076,t1077,t1078,t1079,t1080,t1081,t1082,t1083,t1084,t1085,t1086,t1087,t1088,t1089,t109,t1090,t1091,t1092,t1096,t1097,t1098,t1099,t11,t110,t1100,t1101,t1103,t1104,t1108,t1109,t1110,t1111,t1112,t1113,t1114,t1115,t1116,t1123,t1124,t1125,t1126,t1128,t1129,t113,t1130,t1131,t1132,t1136,t1137,t1138,t1139,t1140,t1141,t1142,t1143,t1144,t1146,t1147,t1148,t1149,t1151,t1152,t1156,t1157,t1158,t1159,t1160,t1161,t1162,t1163,t1164,t1165,t1166,t1167,t1168,t1169,t1170,t1171,t1172,t1173,t1174,t1175,t1176,t1177,t1178,t1179,t118,t1184,t1185,t1186,t1187,t1188,t1189,t1190,t1191,t1193,t1194,t1195,t1197,t1198,t1199,t12,t1200,t1201,t1203,t1204,t1205,t1206,t1207,t1208,t1209,t1210,t1211,t1212,t1214,t1215,t1216,t1217,t1218,t1219,t1220,t1221,t1222,t1223,t1224,t1225,t1226,t1227,t1228,t1229,t123,t1230,t1231,t1232,t1233,t1236,t1237,t1238,t1239,t1240,t1245,t1246,t1247,t1248,t1249,t1253,t1258,t1262,t1263,t1264,t1265,t1266,t1267,t1268,t1269,t1270,t1271,t1272,t1273,t1274,t1275,t1276,t1277,t1278,t1279,t1282,t1284,t1286,t1287,t1288,t1289,t129,t1290,t1291,t1292,t1294,t1296,t1297,t1298,t13,t1300,t1302,t1303,t1304,t1306,t1307,t131,t1310,t1311,t1312,t1313,t1314,t1316,t1317,t1318,t1319,t1322,t1323,t1324,t1325,t1326,t1327,t1328,t1329,t1331,t1332,t1333,t1334,t1335,t1336,t1337,t1338,t1339,t1340,t1341,t1344,t1345,t1346,t1347,t1348,t1349,t1350,t1351,t1352,t1353,t1354,t1355,t1356,t1357,t1358,t1359,t136,t1360,t1361,t1364,t1371,t1372,t1373,t1374,t1376,t1377,t1378,t1380,t1381,t1382,t1384,t1385,t1388,t1389,t1390,t1391,t1392,t1393,t1397,t1400,t1401,t1403,t1404,t1405,t1406,t1410,t1411,t1413,t1414,t1421,t1422,t1423,t1428,t1430,t1432,t1434,t1435,t1436,t1437,t1438,t1439,t144,t1441,t1444,t1445,t1446,t1447,t1448,t1450,t1451,t1452,t1454,t1456,t1457,t1458,t1459,t146,t1461,t1462,t1463,t1466,t1467,t1471,t1474,t1475,t1476,t1477,t1478,t1480,t1483,t1484,t1485,t1486,t1487,t1489,t1491,t1492,t1493,t1495,t1496,t1498,t1503,t1506,t1508,t1509,t1510,t1511,t1512,t1513,t1514,t1516,t1517,t1520,t1521,t1522,t1523,t1524,t1525,t1527,t1528,t1531,t1532,t1533,t1534,t1537,t1538,t1539,t1540,t1542,t1543,t1549,t1550,t1551,t1552,t1553,t16,t160,t1637,t1647,t169,t178,t18,t183,t185,t19,t193,t196,t2,t20,t21,t215,t22,t224,t229,t23,t233,t24,t242,t246,t25,t253,t26,t279,t28,t284,t285,t286,t288,t29,t291,t292,t294,t295,t296,t297,t298,t299,t3,t300,t305,t306,t308,t31,t311,t312,t316,t318,t32,t323,t33,t35,t36,t360,t361,t367,t373,t38,t381,t382,t397,t4,t40,t410,t413,t414,t424,t43,t446,t45,t450,t457,t458,t459,t469,t47,t474,t477,t479,t48,t482,t485,t486,t488,t491,t493,t5,t501,t502,t503,t504,t505,t508,t509,t51,t510,t512,t516,t519,t520,t524,t525,t526,t528,t529,t53,t531,t532,t533,t534,t536,t537,t54,t541,t542,t543,t544,t546,t548,t551,t552,t554,t555,t564,t567,t569,t570,t577,t578,t579,t580,t581,t582,t583,t584,t586,t589,t59,t590,t595,t6,t60,t600,t601,t602,t603,t606,t607,t608,t609,t613,t614,t615,t616,t620,t622,t624,t625,t626,t627,t628,t63,t633,t634,t637,t641,t644,t645,t646,t65,t650,t651,t665,t669,t670,t671,t672,t673,t674,t675,t679,t680,t681,t682,t683,t684,t685,t686,t687,t689,t691,t692,t694,t695,t696,t698,t699,t7,t70,t700,t701,t702,t703,t704,t705,t706,t707,t708,t709,t71,t710,t711,t712,t713,t714,t715,t716,t717,t718,t719,t720,t721,t722,t723,t725,t728,t729,t73,t730,t731,t735,t738,t74,t740,t744,t745,t746,t747,t748,t749,t75,t752,t753,t754,t755,t756,t758,t759,t764,t765,t766,t767,t768,t769,t77,t770,t771,t772,t773,t774,t775,t778,t780,t781,t782,t783,t785,t79,t790,t791,t793,t795,t796,t797,t798,t799,t8,t800,t801,t802,t803,t804,t805,t806,t807,t809,t81,t810,t811,t813,t819,t820,t822,t823,t825,t826,t827,t828,t829,t833,t834,t835,t836,t837,t84,t840,t844,t845,t846,t847,t849,t85,t850,t851,t852,t853,t854,t855,t856,t857,t86,t862,t863,t864,t865,t866,t867,t868,t869,t87,t870,t873,t875,t876,t878,t88,t881,t882,t885,t886,t888,t89,t890,t891,t892,t893,t894,t895,t896,t897,t898,t899,t9,t900,t901,t902,t903,t904,t905,t906,t907,t908,t909,t910,t914,t916,t917,t920,t921,t922,t923,t924,t925,t926,t927,t93,t930,t931,t932,t933,t934,t937,t938,t939,t94,t940,t942,t944,t946,t955,t958,t96,t960,t961,t962,t963,t964,t965,t966,t967,t969,t972,t974,t975,t976,t978,t979,t98,t981,t982,t983,t984,t985,t986,t987,t988,t989,t99,t990,t991,t992,t993,t994,t995,t999});
end
function C = ft_3(ct)
dq1 = ct{1};
dq2 = ct{2};
dq3 = ct{3};
dq4 = ct{4};
dq5 = ct{5};
dq6 = ct{6};
q3 = ct{7};
t10 = ct{8};
t1003 = ct{9};
t1004 = ct{10};
t1005 = ct{11};
t1006 = ct{12};
t1007 = ct{13};
t1008 = ct{14};
t1009 = ct{15};
t101 = ct{16};
t1010 = ct{17};
t1013 = ct{18};
t1014 = ct{19};
t1015 = ct{20};
t1017 = ct{21};
t1018 = ct{22};
t1019 = ct{23};
t102 = ct{24};
t1023 = ct{25};
t1024 = ct{26};
t1027 = ct{27};
t1028 = ct{28};
t1029 = ct{29};
t103 = ct{30};
t1030 = ct{31};
t1031 = ct{32};
t1032 = ct{33};
t1035 = ct{34};
t1036 = ct{35};
t1037 = ct{36};
t1038 = ct{37};
t104 = ct{38};
t1040 = ct{39};
t1041 = ct{40};
t1042 = ct{41};
t1043 = ct{42};
t1044 = ct{43};
t1045 = ct{44};
t1046 = ct{45};
t1047 = ct{46};
t105 = ct{47};
t1053 = ct{48};
t1054 = ct{49};
t1057 = ct{50};
t106 = ct{51};
t1060 = ct{52};
t1061 = ct{53};
t1062 = ct{54};
t1066 = ct{55};
t1067 = ct{56};
t1068 = ct{57};
t1069 = ct{58};
t1070 = ct{59};
t1071 = ct{60};
t1072 = ct{61};
t1073 = ct{62};
t1074 = ct{63};
t1075 = ct{64};
t1076 = ct{65};
t1077 = ct{66};
t1078 = ct{67};
t1079 = ct{68};
t1080 = ct{69};
t1081 = ct{70};
t1082 = ct{71};
t1083 = ct{72};
t1084 = ct{73};
t1085 = ct{74};
t1086 = ct{75};
t1087 = ct{76};
t1088 = ct{77};
t1089 = ct{78};
t109 = ct{79};
t1090 = ct{80};
t1091 = ct{81};
t1092 = ct{82};
t1096 = ct{83};
t1097 = ct{84};
t1098 = ct{85};
t1099 = ct{86};
t11 = ct{87};
t110 = ct{88};
t1100 = ct{89};
t1101 = ct{90};
t1103 = ct{91};
t1104 = ct{92};
t1108 = ct{93};
t1109 = ct{94};
t1110 = ct{95};
t1111 = ct{96};
t1112 = ct{97};
t1113 = ct{98};
t1114 = ct{99};
t1115 = ct{100};
t1116 = ct{101};
t1123 = ct{102};
t1124 = ct{103};
t1125 = ct{104};
t1126 = ct{105};
t1128 = ct{106};
t1129 = ct{107};
t113 = ct{108};
t1130 = ct{109};
t1131 = ct{110};
t1132 = ct{111};
t1136 = ct{112};
t1137 = ct{113};
t1138 = ct{114};
t1139 = ct{115};
t1140 = ct{116};
t1141 = ct{117};
t1142 = ct{118};
t1143 = ct{119};
t1144 = ct{120};
t1146 = ct{121};
t1147 = ct{122};
t1148 = ct{123};
t1149 = ct{124};
t1151 = ct{125};
t1152 = ct{126};
t1156 = ct{127};
t1157 = ct{128};
t1158 = ct{129};
t1159 = ct{130};
t1160 = ct{131};
t1161 = ct{132};
t1162 = ct{133};
t1163 = ct{134};
t1164 = ct{135};
t1165 = ct{136};
t1166 = ct{137};
t1167 = ct{138};
t1168 = ct{139};
t1169 = ct{140};
t1170 = ct{141};
t1171 = ct{142};
t1172 = ct{143};
t1173 = ct{144};
t1174 = ct{145};
t1175 = ct{146};
t1176 = ct{147};
t1177 = ct{148};
t1178 = ct{149};
t1179 = ct{150};
t118 = ct{151};
t1184 = ct{152};
t1185 = ct{153};
t1186 = ct{154};
t1187 = ct{155};
t1188 = ct{156};
t1189 = ct{157};
t1190 = ct{158};
t1191 = ct{159};
t1193 = ct{160};
t1194 = ct{161};
t1195 = ct{162};
t1197 = ct{163};
t1198 = ct{164};
t1199 = ct{165};
t12 = ct{166};
t1200 = ct{167};
t1201 = ct{168};
t1203 = ct{169};
t1204 = ct{170};
t1205 = ct{171};
t1206 = ct{172};
t1207 = ct{173};
t1208 = ct{174};
t1209 = ct{175};
t1210 = ct{176};
t1211 = ct{177};
t1212 = ct{178};
t1214 = ct{179};
t1215 = ct{180};
t1216 = ct{181};
t1217 = ct{182};
t1218 = ct{183};
t1219 = ct{184};
t1220 = ct{185};
t1221 = ct{186};
t1222 = ct{187};
t1223 = ct{188};
t1224 = ct{189};
t1225 = ct{190};
t1226 = ct{191};
t1227 = ct{192};
t1228 = ct{193};
t1229 = ct{194};
t123 = ct{195};
t1230 = ct{196};
t1231 = ct{197};
t1232 = ct{198};
t1233 = ct{199};
t1236 = ct{200};
t1237 = ct{201};
t1238 = ct{202};
t1239 = ct{203};
t1240 = ct{204};
t1245 = ct{205};
t1246 = ct{206};
t1247 = ct{207};
t1248 = ct{208};
t1249 = ct{209};
t1253 = ct{210};
t1258 = ct{211};
t1262 = ct{212};
t1263 = ct{213};
t1264 = ct{214};
t1265 = ct{215};
t1266 = ct{216};
t1267 = ct{217};
t1268 = ct{218};
t1269 = ct{219};
t1270 = ct{220};
t1271 = ct{221};
t1272 = ct{222};
t1273 = ct{223};
t1274 = ct{224};
t1275 = ct{225};
t1276 = ct{226};
t1277 = ct{227};
t1278 = ct{228};
t1279 = ct{229};
t1282 = ct{230};
t1284 = ct{231};
t1286 = ct{232};
t1287 = ct{233};
t1288 = ct{234};
t1289 = ct{235};
t129 = ct{236};
t1290 = ct{237};
t1291 = ct{238};
t1292 = ct{239};
t1294 = ct{240};
t1296 = ct{241};
t1297 = ct{242};
t1298 = ct{243};
t13 = ct{244};
t1300 = ct{245};
t1302 = ct{246};
t1303 = ct{247};
t1304 = ct{248};
t1306 = ct{249};
t1307 = ct{250};
t131 = ct{251};
t1310 = ct{252};
t1311 = ct{253};
t1312 = ct{254};
t1313 = ct{255};
t1314 = ct{256};
t1316 = ct{257};
t1317 = ct{258};
t1318 = ct{259};
t1319 = ct{260};
t1322 = ct{261};
t1323 = ct{262};
t1324 = ct{263};
t1325 = ct{264};
t1326 = ct{265};
t1327 = ct{266};
t1328 = ct{267};
t1329 = ct{268};
t1331 = ct{269};
t1332 = ct{270};
t1333 = ct{271};
t1334 = ct{272};
t1335 = ct{273};
t1336 = ct{274};
t1337 = ct{275};
t1338 = ct{276};
t1339 = ct{277};
t1340 = ct{278};
t1341 = ct{279};
t1344 = ct{280};
t1345 = ct{281};
t1346 = ct{282};
t1347 = ct{283};
t1348 = ct{284};
t1349 = ct{285};
t1350 = ct{286};
t1351 = ct{287};
t1352 = ct{288};
t1353 = ct{289};
t1354 = ct{290};
t1355 = ct{291};
t1356 = ct{292};
t1357 = ct{293};
t1358 = ct{294};
t1359 = ct{295};
t136 = ct{296};
t1360 = ct{297};
t1361 = ct{298};
t1364 = ct{299};
t1371 = ct{300};
t1372 = ct{301};
t1373 = ct{302};
t1374 = ct{303};
t1376 = ct{304};
t1377 = ct{305};
t1378 = ct{306};
t1380 = ct{307};
t1381 = ct{308};
t1382 = ct{309};
t1384 = ct{310};
t1385 = ct{311};
t1388 = ct{312};
t1389 = ct{313};
t1390 = ct{314};
t1391 = ct{315};
t1392 = ct{316};
t1393 = ct{317};
t1397 = ct{318};
t1400 = ct{319};
t1401 = ct{320};
t1403 = ct{321};
t1404 = ct{322};
t1405 = ct{323};
t1406 = ct{324};
t1410 = ct{325};
t1411 = ct{326};
t1413 = ct{327};
t1414 = ct{328};
t1421 = ct{329};
t1422 = ct{330};
t1423 = ct{331};
t1428 = ct{332};
t1430 = ct{333};
t1432 = ct{334};
t1434 = ct{335};
t1435 = ct{336};
t1436 = ct{337};
t1437 = ct{338};
t1438 = ct{339};
t1439 = ct{340};
t144 = ct{341};
t1441 = ct{342};
t1444 = ct{343};
t1445 = ct{344};
t1446 = ct{345};
t1447 = ct{346};
t1448 = ct{347};
t1450 = ct{348};
t1451 = ct{349};
t1452 = ct{350};
t1454 = ct{351};
t1456 = ct{352};
t1457 = ct{353};
t1458 = ct{354};
t1459 = ct{355};
t146 = ct{356};
t1461 = ct{357};
t1462 = ct{358};
t1463 = ct{359};
t1466 = ct{360};
t1467 = ct{361};
t1471 = ct{362};
t1474 = ct{363};
t1475 = ct{364};
t1476 = ct{365};
t1477 = ct{366};
t1478 = ct{367};
t1480 = ct{368};
t1483 = ct{369};
t1484 = ct{370};
t1485 = ct{371};
t1486 = ct{372};
t1487 = ct{373};
t1489 = ct{374};
t1491 = ct{375};
t1492 = ct{376};
t1493 = ct{377};
t1495 = ct{378};
t1496 = ct{379};
t1498 = ct{380};
t1503 = ct{381};
t1506 = ct{382};
t1508 = ct{383};
t1509 = ct{384};
t1510 = ct{385};
t1511 = ct{386};
t1512 = ct{387};
t1513 = ct{388};
t1514 = ct{389};
t1516 = ct{390};
t1517 = ct{391};
t1520 = ct{392};
t1521 = ct{393};
t1522 = ct{394};
t1523 = ct{395};
t1524 = ct{396};
t1525 = ct{397};
t1527 = ct{398};
t1528 = ct{399};
t1531 = ct{400};
t1532 = ct{401};
t1533 = ct{402};
t1534 = ct{403};
t1537 = ct{404};
t1538 = ct{405};
t1539 = ct{406};
t1540 = ct{407};
t1542 = ct{408};
t1543 = ct{409};
t1549 = ct{410};
t1550 = ct{411};
t1551 = ct{412};
t1552 = ct{413};
t1553 = ct{414};
t16 = ct{415};
t160 = ct{416};
t1637 = ct{417};
t1647 = ct{418};
t169 = ct{419};
t178 = ct{420};
t18 = ct{421};
t183 = ct{422};
t185 = ct{423};
t19 = ct{424};
t193 = ct{425};
t196 = ct{426};
t2 = ct{427};
t20 = ct{428};
t21 = ct{429};
t215 = ct{430};
t22 = ct{431};
t224 = ct{432};
t229 = ct{433};
t23 = ct{434};
t233 = ct{435};
t24 = ct{436};
t242 = ct{437};
t246 = ct{438};
t25 = ct{439};
t253 = ct{440};
t26 = ct{441};
t279 = ct{442};
t28 = ct{443};
t284 = ct{444};
t285 = ct{445};
t286 = ct{446};
t288 = ct{447};
t29 = ct{448};
t291 = ct{449};
t292 = ct{450};
t294 = ct{451};
t295 = ct{452};
t296 = ct{453};
t297 = ct{454};
t298 = ct{455};
t299 = ct{456};
t3 = ct{457};
t300 = ct{458};
t305 = ct{459};
t306 = ct{460};
t308 = ct{461};
t31 = ct{462};
t311 = ct{463};
t312 = ct{464};
t316 = ct{465};
t318 = ct{466};
t32 = ct{467};
t323 = ct{468};
t33 = ct{469};
t35 = ct{470};
t36 = ct{471};
t360 = ct{472};
t361 = ct{473};
t367 = ct{474};
t373 = ct{475};
t38 = ct{476};
t381 = ct{477};
t382 = ct{478};
t397 = ct{479};
t4 = ct{480};
t40 = ct{481};
t410 = ct{482};
t413 = ct{483};
t414 = ct{484};
t424 = ct{485};
t43 = ct{486};
t446 = ct{487};
t45 = ct{488};
t450 = ct{489};
t457 = ct{490};
t458 = ct{491};
t459 = ct{492};
t469 = ct{493};
t47 = ct{494};
t474 = ct{495};
t477 = ct{496};
t479 = ct{497};
t48 = ct{498};
t482 = ct{499};
t485 = ct{500};
t486 = ct{501};
t488 = ct{502};
t491 = ct{503};
t493 = ct{504};
t5 = ct{505};
t501 = ct{506};
t502 = ct{507};
t503 = ct{508};
t504 = ct{509};
t505 = ct{510};
t508 = ct{511};
t509 = ct{512};
t51 = ct{513};
t510 = ct{514};
t512 = ct{515};
t516 = ct{516};
t519 = ct{517};
t520 = ct{518};
t524 = ct{519};
t525 = ct{520};
t526 = ct{521};
t528 = ct{522};
t529 = ct{523};
t53 = ct{524};
t531 = ct{525};
t532 = ct{526};
t533 = ct{527};
t534 = ct{528};
t536 = ct{529};
t537 = ct{530};
t54 = ct{531};
t541 = ct{532};
t542 = ct{533};
t543 = ct{534};
t544 = ct{535};
t546 = ct{536};
t548 = ct{537};
t551 = ct{538};
t552 = ct{539};
t554 = ct{540};
t555 = ct{541};
t564 = ct{542};
t567 = ct{543};
t569 = ct{544};
t570 = ct{545};
t577 = ct{546};
t578 = ct{547};
t579 = ct{548};
t580 = ct{549};
t581 = ct{550};
t582 = ct{551};
t583 = ct{552};
t584 = ct{553};
t586 = ct{554};
t589 = ct{555};
t59 = ct{556};
t590 = ct{557};
t595 = ct{558};
t6 = ct{559};
t60 = ct{560};
t600 = ct{561};
t601 = ct{562};
t602 = ct{563};
t603 = ct{564};
t606 = ct{565};
t607 = ct{566};
t608 = ct{567};
t609 = ct{568};
t613 = ct{569};
t614 = ct{570};
t615 = ct{571};
t616 = ct{572};
t620 = ct{573};
t622 = ct{574};
t624 = ct{575};
t625 = ct{576};
t626 = ct{577};
t627 = ct{578};
t628 = ct{579};
t63 = ct{580};
t633 = ct{581};
t634 = ct{582};
t637 = ct{583};
t641 = ct{584};
t644 = ct{585};
t645 = ct{586};
t646 = ct{587};
t65 = ct{588};
t650 = ct{589};
t651 = ct{590};
t665 = ct{591};
t669 = ct{592};
t670 = ct{593};
t671 = ct{594};
t672 = ct{595};
t673 = ct{596};
t674 = ct{597};
t675 = ct{598};
t679 = ct{599};
t680 = ct{600};
t681 = ct{601};
t682 = ct{602};
t683 = ct{603};
t684 = ct{604};
t685 = ct{605};
t686 = ct{606};
t687 = ct{607};
t689 = ct{608};
t691 = ct{609};
t692 = ct{610};
t694 = ct{611};
t695 = ct{612};
t696 = ct{613};
t698 = ct{614};
t699 = ct{615};
t7 = ct{616};
t70 = ct{617};
t700 = ct{618};
t701 = ct{619};
t702 = ct{620};
t703 = ct{621};
t704 = ct{622};
t705 = ct{623};
t706 = ct{624};
t707 = ct{625};
t708 = ct{626};
t709 = ct{627};
t71 = ct{628};
t710 = ct{629};
t711 = ct{630};
t712 = ct{631};
t713 = ct{632};
t714 = ct{633};
t715 = ct{634};
t716 = ct{635};
t717 = ct{636};
t718 = ct{637};
t719 = ct{638};
t720 = ct{639};
t721 = ct{640};
t722 = ct{641};
t723 = ct{642};
t725 = ct{643};
t728 = ct{644};
t729 = ct{645};
t73 = ct{646};
t730 = ct{647};
t731 = ct{648};
t735 = ct{649};
t738 = ct{650};
t74 = ct{651};
t740 = ct{652};
t744 = ct{653};
t745 = ct{654};
t746 = ct{655};
t747 = ct{656};
t748 = ct{657};
t749 = ct{658};
t75 = ct{659};
t752 = ct{660};
t753 = ct{661};
t754 = ct{662};
t755 = ct{663};
t756 = ct{664};
t758 = ct{665};
t759 = ct{666};
t764 = ct{667};
t765 = ct{668};
t766 = ct{669};
t767 = ct{670};
t768 = ct{671};
t769 = ct{672};
t77 = ct{673};
t770 = ct{674};
t771 = ct{675};
t772 = ct{676};
t773 = ct{677};
t774 = ct{678};
t775 = ct{679};
t778 = ct{680};
t780 = ct{681};
t781 = ct{682};
t782 = ct{683};
t783 = ct{684};
t785 = ct{685};
t79 = ct{686};
t790 = ct{687};
t791 = ct{688};
t793 = ct{689};
t795 = ct{690};
t796 = ct{691};
t797 = ct{692};
t798 = ct{693};
t799 = ct{694};
t8 = ct{695};
t800 = ct{696};
t801 = ct{697};
t802 = ct{698};
t803 = ct{699};
t804 = ct{700};
t805 = ct{701};
t806 = ct{702};
t807 = ct{703};
t809 = ct{704};
t81 = ct{705};
t810 = ct{706};
t811 = ct{707};
t813 = ct{708};
t819 = ct{709};
t820 = ct{710};
t822 = ct{711};
t823 = ct{712};
t825 = ct{713};
t826 = ct{714};
t827 = ct{715};
t828 = ct{716};
t829 = ct{717};
t833 = ct{718};
t834 = ct{719};
t835 = ct{720};
t836 = ct{721};
t837 = ct{722};
t84 = ct{723};
t840 = ct{724};
t844 = ct{725};
t845 = ct{726};
t846 = ct{727};
t847 = ct{728};
t849 = ct{729};
t85 = ct{730};
t850 = ct{731};
t851 = ct{732};
t852 = ct{733};
t853 = ct{734};
t854 = ct{735};
t855 = ct{736};
t856 = ct{737};
t857 = ct{738};
t86 = ct{739};
t862 = ct{740};
t863 = ct{741};
t864 = ct{742};
t865 = ct{743};
t866 = ct{744};
t867 = ct{745};
t868 = ct{746};
t869 = ct{747};
t87 = ct{748};
t870 = ct{749};
t873 = ct{750};
t875 = ct{751};
t876 = ct{752};
t878 = ct{753};
t88 = ct{754};
t881 = ct{755};
t882 = ct{756};
t885 = ct{757};
t886 = ct{758};
t888 = ct{759};
t89 = ct{760};
t890 = ct{761};
t891 = ct{762};
t892 = ct{763};
t893 = ct{764};
t894 = ct{765};
t895 = ct{766};
t896 = ct{767};
t897 = ct{768};
t898 = ct{769};
t899 = ct{770};
t9 = ct{771};
t900 = ct{772};
t901 = ct{773};
t902 = ct{774};
t903 = ct{775};
t904 = ct{776};
t905 = ct{777};
t906 = ct{778};
t907 = ct{779};
t908 = ct{780};
t909 = ct{781};
t910 = ct{782};
t914 = ct{783};
t916 = ct{784};
t917 = ct{785};
t920 = ct{786};
t921 = ct{787};
t922 = ct{788};
t923 = ct{789};
t924 = ct{790};
t925 = ct{791};
t926 = ct{792};
t927 = ct{793};
t93 = ct{794};
t930 = ct{795};
t931 = ct{796};
t932 = ct{797};
t933 = ct{798};
t934 = ct{799};
t937 = ct{800};
t938 = ct{801};
t939 = ct{802};
t94 = ct{803};
t940 = ct{804};
t942 = ct{805};
t944 = ct{806};
t946 = ct{807};
t955 = ct{808};
t958 = ct{809};
t96 = ct{810};
t960 = ct{811};
t961 = ct{812};
t962 = ct{813};
t963 = ct{814};
t964 = ct{815};
t965 = ct{816};
t966 = ct{817};
t967 = ct{818};
t969 = ct{819};
t972 = ct{820};
t974 = ct{821};
t975 = ct{822};
t976 = ct{823};
t978 = ct{824};
t979 = ct{825};
t98 = ct{826};
t981 = ct{827};
t982 = ct{828};
t983 = ct{829};
t984 = ct{830};
t985 = ct{831};
t986 = ct{832};
t987 = ct{833};
t988 = ct{834};
t989 = ct{835};
t99 = ct{836};
t990 = ct{837};
t991 = ct{838};
t992 = ct{839};
t993 = ct{840};
t994 = ct{841};
t995 = ct{842};
t999 = ct{843};
t1554 = t11.*t1543;
t1555 = t1444.*1.0e-1;
t1567 = t850.*t1520;
t1571 = t1046.*t1522;
t1573 = t1045.*t1532;
t1574 = t850.*t1543;
t1575 = t1323.*t1503;
t1578 = t1046.*t1542;
t1588 = t1326.*t1514;
t1591 = t1325.*t1512;
t1595 = t1317.*t1522;
t1597 = t1316.*t1532;
t1598 = t1316.*t1534;
t1604 = t1322.*t1543;
t1612 = t1372.*t1522;
t1617 = t1371.*t1532;
t1624 = t1372.*t1542;
t1627 = t1384.*t1520;
t1636 = t1384.*t1543;
t1639 = t1405+t1422+t1430;
t1675 = t224+t825+t826+t827+t940+t942+t944+t1023+t1024+t1146+t1147+t1148+t1149;
t1676 = t242+t828+t829+t837+t840+t930+t946+t1027+t1028+t1029+t1151+t1152+t1247;
t1683 = t1522.*t1542;
t1684 = t1520.*t1543;
t1704 = t479+t485+t488+t503+t508+t516+t519+t524+t536+t544+t600+t622+t699+t701+t703+t705+t711+t712+t715+t716+t852+t895;
t1706 = t486+t491+t493+t510+t512+t525+t531+t533+t548+t552+t603+t624+t684+t685+t686+t687+t694+t695+t696+t868+t869+t870;
t1710 = t520+t526+t529+t542+t546+t564+t601+t606+t607+t728+t729+t730+t731+t735+t738+t740+t744+t745+t746+t855+t856+t857;
t1711 = t469+t474+t477+t482+t501+t504+t613+t614+t620+t680+t681+t682+t683+t689+t691+t692+t764+t765+t766+t865+t866+t867;
t1712 = t502+t505+t509+t537+t541+t543+t698+t700+t702+t704+t710+t713+t714+t717+t722+t723+t725+t778+t780+t781+t853+t894;
t1770 = t311+t312+t885+t886+t888+t906+t907+t909+t1083+t1084+t1085+t1086+t1166+t1184+t1185+t1186+t1198+t1199+t1200+t1201+t1230+t1231+t1232+t1233+t1262+t1287+t1288;
t1771 = t253+t318+t908+t910+t914+t987+t1009+t1010+t1108+t1109+t1110+t1130+t1131+t1132+t1177+t1178+t1179+t1193+t1194+t1195+t1237+t1238+t1239+t1240+t1278+t1290+t1291;
t1776 = t323+t569+t625+t626+t634+t675+t754+t756+t758+t759+t773+t774+t864+t873+t875+t876+t878+t881+t882+t901+t903+t905+t916+t917+t960+t962+t963+t1057+t1060+t1061+t1062+t1112+t1113+t1115;
t1778 = t279+t459+t580+t581+t584+t586+t589+t590+t650+t651+t673+t679+t793+t800+t802+t803+t804+t805+t807+t810+t813+t819+t820+t822+t823+t920+t924+t933+t934+t938+t1017+t1018+t1019+t1143+t1144;
t1779 = t457+t458+t577+t578+t579+t582+t583+t669+t670+t671+t672+t674+t790+t791+t795+t796+t797+t798+t799+t801+t806+t809+t811+t833+t925+t926+t927+t931+t932+t939+t1138+t1139+t1140+t1141+t1142;
t1802 = t615+t616+t633+t752+t753+t755+t767+t768+t770+t772+t775+t844+t863+t900+t902+t904+t921+t922+t955+t958+t961+t964+t965+t966+t967+t969+t972+t975+t976+t979+t981+t984+t985+t986+t991+t992+t993+t1013+t1014+t1015+t1031+t1032+t1053+t1070+t1073+t1074+t1075+t1076+t1077+t1078+t1100+t1101+t1103+t1104+t1111+t1114+t1116+t1128+t1156+t1157+t1158+t1159+t1160+t1161+t1162+t1163+t1164+t1165+t1187+t1188+t1189+t1190+t1212+t1217+t1218+t1219+t1220+t1221+t1227+t1228+t1229;
t1803 = t570+t627+t628+t769+t771+t782+t783+t785+t862+t890+t891+t892+t893+t897+t898+t899+t923+t937+t974+t978+t982+t983+t988+t989+t990+t994+t995+t999+t1003+t1004+t1005+t1006+t1007+t1008+t1037+t1038+t1054+t1066+t1067+t1068+t1069+t1071+t1072+t1079+t1080+t1081+t1082+t1087+t1088+t1089+t1090+t1091+t1092+t1096+t1097+t1098+t1099+t1123+t1124+t1125+t1126+t1129+t1167+t1168+t1169+t1170+t1171+t1172+t1173+t1174+t1175+t1176+t1214+t1215+t1216+t1222+t1223+t1224+t1225+t1226+t1236;
t1293 = -t1263;
t1309 = t16.*t1292;
t1320 = -t1312;
t1365 = -t1348;
t1366 = -t1350;
t1367 = -t1353;
t1368 = -t1356;
t1369 = -t1358;
t1370 = t1357./1.0e+1;
t1386 = t1286+t1289;
t1394 = -t1389;
t1395 = -t1390;
t1398 = -t1392;
t1408 = dq6.*t1400.*2.0;
t1409 = dq6.*t1403.*2.0;
t1416 = -t1400;
t1417 = -t1404;
t1429 = -t1421;
t1431 = t1413./1.0e+1;
t1433 = t1292+t1341;
t1440 = t1436./1.0e+1;
t1442 = -t1438;
t1443 = t1441./1.0e+1;
t1455 = -t1447;
t1465 = -t1454;
t1469 = -t1458;
t1470 = -t1459;
t1479 = t1456./1.0e+1;
t1481 = -t1480;
t1482 = -t1476;
t1488 = -t1487;
t1490 = -t1486;
t1494 = t1486./1.0e+1;
t1499 = t1489./1.0e+1;
t1500 = t1491./1.0e+1;
t1504 = t1492./1.0e+1;
t1505 = t1493./1.0e+1;
t1507 = t1498./1.0e+1;
t1515 = t1316.*t1451;
t1519 = -t1516;
t1526 = t1316.*t1474;
t1529 = t1438.*1.0e-1;
t1530 = t1439.*1.0e-1;
t1535 = -t1524;
t1541 = -t1528;
t1544 = dq6.*t1539.*2.0;
t1545 = dq6.*t1540.*2.0;
t1546 = -t1540;
t1548 = t1533./1.0e+1;
t1556 = t850.*t1510;
t1557 = -t1550;
t1558 = dq6.*t1552.*2.0;
t1559 = dq6.*t1554.*2.0;
t1560 = t1550./1.0e+1;
t1561 = t1447.*1.0e-1;
t1565 = t1458.*1.0e-1;
t1566 = t1459.*1.0e-1;
t1568 = t1045.*t1517;
t1572 = t1567./1.0e+1;
t1576 = t1045.*t1531;
t1577 = t1411.*t1448;
t1579 = -t1574;
t1580 = t1571./1.0e+1;
t1581 = t1428.*t1450;
t1582 = t1428.*t1452;
t1584 = t1574./1.0e+1;
t1587 = t1411.*t1471;
t1589 = t1485.*1.0e-1;
t1590 = t1578./1.0e+1;
t1596 = -t1591;
t1600 = t1591./1.0e+1;
t1601 = t1496.*1.0e-1;
t1603 = -t1597;
t1605 = t1506.*1.0e-1;
t1606 = t1249+t1436+t1441;
t1607 = t1351+t1537;
t1608 = t1364+t1538;
t1609 = t1337+t1553;
t1611 = t1516.*1.0e-1;
t1613 = t1355+t1551;
t1616 = t1371.*t1531;
t1618 = t646+t1297+t1349+t1475;
t1620 = t1525.*1.0e-1;
t1622 = t1527.*1.0e-1;
t1623 = t1528.*1.0e-1;
t1629 = t410+t413+t644+t646+t1297+t1475;
t1630 = t382+t1311+t1352+t1483;
t1632 = -t1627;
t1633 = t1617./1.0e+1;
t1634 = t414+t424+t641+t645+t1298+t1484;
t1635 = t360+t373+t382+t665+t1311+t1483;
t1638 = t1624./1.0e+1;
t1641 = t1627./1.0e+1;
t1642 = t1549.*1.0e-1;
t1643 = t1411.*t1520;
t1645 = t1428.*t1522;
t1646 = t1411.*t1543;
t1650 = t1428.*t1542;
t1656 = t1573.*1.0e-1;
t1657 = t1575.*1.0e-1;
t1659 = t1264+t1314+t1393+t1477;
t1661 = t1588.*1.0e-1;
t1664 = t1595.*1.0e-1;
t1665 = t1597.*1.0e-1;
t1666 = t1598.*1.0e-1;
t1669 = t1604.*1.0e-1;
t1670 = t1612.*1.0e-1;
t1673 = t1636.*1.0e-1;
t1674 = -t1317.*(t1203-t1313+t1404-t1466);
t1678 = t1317.*(t1203-t1313+t1404-t1466);
t1682 = t1204+t1354+t1403+t1552;
t1685 = t1531.*t1532;
t1686 = -t1684;
t1689 = (t1258-t1341).*(t1206+t1312-t1401-t1467);
t1690 = -t1317.*(t1263+t1356-t1381-t1539);
t1699 = t1683.*1.0e-1;
t1700 = t1684.*1.0e-1;
t1709 = t528+t532+t534+t551+t554+t567+t602+t608+t609+t706+t707+t708+t709+t718+t719+t720+t721+t747+t748+t749+t854+t896;
t1713 = t6.*t1710;
t1714 = t11.*t1710;
t1715 = t1317.*(t1263+t1356-t1381-t1539).*(-1.0e-1);
t1717 = t6.*t1712;
t1718 = t11.*t1712;
t1721 = t1046.*t1704;
t1722 = t1045.*t1706;
t1727 = t850.*t1711;
t1728 = t1391+t1567+t1578;
t1733 = t1317.*t1710;
t1736 = t1322.*t1712;
t1742 = -t1542.*(t1263+t1356-t1381-t1539);
t1744 = t1542.*(t1263+t1356-t1381-t1539);
t1745 = t1428.*t1704;
t1750 = t1411.*t1711;
t1754 = t1439+t1595+t1604;
t1419 = -t1408;
t1497 = -t1494;
t1518 = -t1515;
t1536 = -t1529;
t1547 = -t1544;
t1562 = -t1560;
t1563 = -t1561;
t1564 = t1556./1.0e+1;
t1569 = -t1565;
t1570 = -t1566;
t1583 = -t1577;
t1585 = -t1584;
t1586 = t1577./1.0e+1;
t1593 = t1581./1.0e+1;
t1594 = t1582./1.0e+1;
t1599 = t1587./1.0e+1;
t1602 = -t1600;
t1610 = t1515.*1.0e-1;
t1615 = -t1611;
t1619 = t381+t1296+t1345+t1482;
t1621 = t1526.*1.0e-1;
t1625 = -t1623;
t1626 = -t1616;
t1628 = t361+t367+t381+t637+t1296+t1482;
t1631 = t424+t1298+t1365+t1484;
t1640 = t1306+t1440+t1443;
t1644 = -t1641;
t1648 = -t1645;
t1649 = t1643./1.0e+1;
t1651 = t1645./1.0e+1;
t1652 = t1568.*1.0e-1;
t1654 = t1646./1.0e+1;
t1655 = t1650./1.0e+1;
t1658 = t1576.*1.0e-1;
t1660 = t1269+t1300+t1398+t1478;
t1662 = t1270+t1320+t1401+t1467;
t1663 = t1265+t1313+t1417+t1466;
t1667 = -t1665;
t1668 = t1339+t1444+t1469;
t1671 = t1616.*1.0e-1;
t1677 = t1322.*t1659;
t1680 = t1293+t1368+t1381+t1539;
t1681 = t1268+t1367+t1380+t1546;
t1687 = t1207+t1366+t1416+t1554;
t1692 = t1322.*t1682;
t1693 = t1678.*(-1.0e-1);
t1695 = t1678.*1.0e-1;
t1701 = t1685.*1.0e-1;
t1702 = -t1700;
t1708 = t1689.*1.0e-1;
t1719 = -t1718;
t1723 = -t1722;
t1725 = t1721./1.0e+1;
t1729 = -t1727;
t1730 = t1727./1.0e+1;
t1732 = t1316.*t1709;
t1734 = t1410+t1572+t1590;
t1735 = -t1733;
t1739 = -t1736;
t1741 = t1520.*t1682;
t1748 = t1745./1.0e+1;
t1751 = t1722.*1.0e-1;
t1752 = -t1750;
t1755 = t1750./1.0e+1;
t1758 = t1733.*1.0e-1;
t1760 = t1736.*1.0e-1;
t1763 = t1744.*(-1.0e-1);
t1764 = t1744.*1.0e-1;
t1765 = t1446+t1643+t1650;
t1772 = t1530+t1664+t1669;
t1777 = t1279+t1302+t1357+t1489+t1490+t1556+t1557;
t1784 = t1309+t1359+t1394+t1535+t1545+t1713;
t1790 = t1388+t1442+t1575+t1588+t1612+t1636;
t1592 = -t1586;
t1614 = -t1610;
t1653 = -t1651;
t1672 = -t1671;
t1679 = -t1677;
t1688 = -t1660.*(t1197-t1340);
t1691 = t1317.*t1681;
t1694 = t1677.*1.0e-1;
t1696 = t1322.*t1687;
t1703 = -t1681.*(t1258-t1341);
t1705 = t1660.*(t1197-t1340).*(-1.0e-1);
t1707 = -t1687.*(t1197-t1340);
t1720 = t1692.*1.0e-1;
t1731 = -t1730;
t1737 = t1462+t1555+t1569;
t1738 = t1681.*(t1258-t1341).*(-1.0e-1);
t1740 = t1687.*(t1197-t1340).*(-1.0e-1);
t1743 = t1542.*t1681;
t1746 = t1520.*t1687;
t1753 = -t1751;
t1756 = -t1755;
t1757 = t1732.*1.0e-1;
t1759 = -t1758;
t1761 = -t1760;
t1762 = t1741.*1.0e-1;
t1766 = t1465+t1649+t1655;
t1767 = -t1681.*(t1263+t1356-t1381-t1539);
t1768 = t1682.*t1687;
t1773 = t1681.*(t1263+t1356-t1381-t1539).*(-1.0e-1);
t1780 = t1310+t1318+t1370+t1497+t1499+t1562+t1564;
t1781 = t1294+t1361+t1395+t1523+t1547+t1714;
t1782 = t1276+t1360+t1409+t1508+t1558+t1719;
t1783 = t1576+t1690+t1692;
t1785 = t1277+t1369+t1419+t1509+t1559+t1717;
t1786 = t1317.*t1784;
t1798 = t1488+t1536+t1657+t1661+t1670+t1673;
t1799 = t1397+t1406+t1533+t1624+t1632+t1721+t1729;
t1801 = t1485+t1549+t1683+t1686+t1735+t1739;
t1697 = -t1694;
t1698 = -t1696;
t1716 = t1691.*1.0e-1;
t1724 = t1696.*1.0e-1;
t1747 = t1743./1.0e+1;
t1749 = t1746./1.0e+1;
t1769 = -t1768;
t1774 = t1768.*1.0e-1;
t1787 = t1322.*t1785;
t1788 = -t1781.*(t1258-t1341);
t1789 = -t1782.*(t1197-t1340);
t1791 = t1603+t1703+t1707;
t1792 = t1786.*1.0e-1;
t1794 = t1781.*(t1258-t1341).*(-1.0e-1);
t1795 = t1782.*(t1197-t1340).*(-1.0e-1);
t1796 = t1658+t1715+t1720;
t1797 = t1667+t1738+t1740;
t1800 = t1423+t1429+t1548+t1638+t1644+t1725+t1731;
t1804 = t1589+t1642+t1699+t1702+t1759+t1761;
t1805 = t1596+t1617+t1743+t1745+t1746+t1752;
t1726 = -t1724;
t1775 = -t1774;
t1793 = t1787.*1.0e-1;
t1806 = t1602+t1633+t1747+t1748+t1749+t1756;
t1807 = t1626+t1723+t1741+t1744+t1786+t1787;
t1809 = t1685+t1732+t1767+t1769+t1788+t1789;
t1808 = t1672+t1753+t1762+t1764+t1792+t1793;
t1810 = t1701+t1757+t1773+t1775+t1794+t1795;
et1 = t1597+t1687.*(t1197-t1340)+t1681.*(t1258-t1341);
et2 = (t1428.*t1682.*1.0e-1-t1681.*(t1197-t1340).*1.0e-1+t1687.*(t1258-t1341).*1.0e-1-t1411.*(t1263+t1356-t1381-t1539).*1.0e-1).*(-1.0./2.0);
et3 = (t1803.*(t73.*9.1e+1+t77.*9.1e+1-t292.*9.1e+1-t2.*t3.*1.56e+2-t11.*t32.*1.0e+2+t6.*t73.*1.0e+2+t6.*t77.*1.0e+2-t11.*t98.*1.0e+2-t28.*t110.*1.0e+2+q3.*t2.*t3.*1.0e+4))./1.0e+10+(t1802.*(t87.*-9.1e+1+t103.*9.1e+1+t306.*9.1e+1+t3.*t7.*1.56e+2-t11.*t28.*1.0e+2+t11.*t71.*1.0e+2-t7.*t81.*1.0e+2+t6.*t103.*1.0e+2+t32.*t110.*1.0e+2-q3.*t3.*t7.*1.0e+4))./1.0e+10-(t1808.*(t1317.*(t1197-t1340)+t1322.*(t1258-t1341)))./2.0;
et4 = t1807.*(t1317.*(t1197-t1340).*1.0e-1+t1322.*(t1258-t1341).*1.0e-1).*(-1.0./2.0)+(t1796.*(t1317.*t1682+t1542.*(t1197-t1340)-t1520.*(t1258-t1341)+t1322.*(t1263+t1356-t1381-t1539)))./2.0;
et5 = (t1783.*(t1317.*t1682.*1.0e-1+t1542.*(t1197-t1340).*1.0e-1-t1520.*(t1258-t1341).*1.0e-1+t1322.*(t1263+t1356-t1381-t1539).*1.0e-1))./2.0;
et6 = dq2.*t26.*(7.0./5.0e+2)+t3.*t13.*3.2774e-3+t8.*t13.*1.79e-3-t54.*t595.*5.0e-2-t59.*t595.*5.0e-2-t45.*t851.*5.0e-2;
et7 = t65.*t851.*5.0e-2+(t40.*t1376)./1.0e+2+(t51.*t1374)./1.0e+2-(t45.*t1513)./2.0-(t54.*t1511)./2.0-(t59.*t1511)./2.0+(t65.*t1513)./2.0+(t1030.*t1374)./1.0e+2-(t1035.*t1376)./1.0e+2-(t1036.*t1376)./1.0e+2-(t1043.*t1374)./1.0e+2+(t1640.*(t849.*t1384+t850.*t1385-t1046.*t1373+t1047.*t1372))./2.0+(t1606.*((t849.*t1384)./1.0e+1+(t850.*t1385)./1.0e+1-(t1046.*t1373)./1.0e+1+(t1047.*t1372)./1.0e+1))./2.0+(t1734.*(t850.*t1542-t1046.*t1520-t1322.*t1372+t1317.*t1384))./2.0;
et8 = (t1737.*(t850.*t1522+t1046.*t1543+t1323.*t1372+t1326.*t1384))./2.0+(t1728.*((t850.*t1542)./1.0e+1-(t1046.*t1520)./1.0e+1-(t1322.*t1372)./1.0e+1+(t1317.*t1384)./1.0e+1))./2.0-(t1772.*(t1322.*t1522-t1326.*t1520-t1317.*t1543+t1323.*t1542))./2.0-(t1766.*(t1428.*t1520-t1411.*t1542+t1322.*t1681+t1317.*t1687))./2.0-(t1765.*((t1428.*t1520)./1.0e+1-(t1411.*t1542)./1.0e+1+(t1322.*t1681)./1.0e+1+(t1317.*t1687)./1.0e+1))./2.0;
et9 = (t1668.*(t850.*t1522.*1.0e-1+t1046.*t1543.*1.0e-1+t1323.*t1372.*1.0e-1+t1326.*t1384.*1.0e-1))./2.0;
et10 = t1754.*(t1322.*t1522.*1.0e-1-t1326.*t1520.*1.0e-1-t1317.*t1543.*1.0e-1+t1323.*t1542.*1.0e-1).*(-1.0./2.0);
et11 = (t1771.*(t73./1.0e+2+t77./1.0e+2-t292./1.0e+2+t2.*t3.*t555))./1.0e+2-(t1770.*(t87./1.0e+2-t103./1.0e+2-t306./1.0e+2+t3.*t7.*t555))./1.0e+2;
et12 = (t1665+t1687.*(t1197-t1340).*1.0e-1+t1681.*(t1258-t1341).*1.0e-1).*(t1428.*t1682-t1681.*(t1197-t1340)+t1687.*(t1258-t1341)-t1411.*(t1263+t1356-t1381-t1539)).*(-1.0./2.0)+et1.*et2+(t1780.*(t849.*t850-t1046.*t1047))./2.0+(t1777.*((t849.*t850)./1.0e+1-(t1046.*t1047)./1.0e+1))./2.0-(t1800.*(t850.*t1317+t1046.*t1322))./2.0;
et13 = (t1798.*(t850.*t1326-t1046.*t1323))./2.0-(t1799.*((t850.*t1317)./1.0e+1+(t1046.*t1322)./1.0e+1))./2.0-(t1804.*(t1317.*t1323+t1322.*t1326))./2.0+(t1790.*(t850.*t1326.*1.0e-1-t1046.*t1323.*1.0e-1))./2.0-(t1806.*(t1317.*t1411+t1322.*t1428))./2.0-(t1805.*((t1317.*t1411)./1.0e+1+(t1322.*t1428)./1.0e+1))./2.0;
et14 = t1801.*(t1317.*t1323.*1.0e-1+t1322.*t1326.*1.0e-1).*(-1.0./2.0);
et15 = (t1428.*(t1197-t1340).*1.0e-1-t1411.*(t1258-t1341).*1.0e-1).*(-t1685-t1732+t1768+t1782.*(t1197-t1340)+t1781.*(t1258-t1341)+t1681.*(t1263+t1356-t1381-t1539)).*(-1.0./2.0);
et16 = (t1428.*(t1197-t1340)-t1411.*(t1258-t1341)).*(-t1701-t1757+t1774+t1782.*(t1197-t1340).*1.0e-1+t1781.*(t1258-t1341).*1.0e-1+t1681.*(t1263+t1356-t1381-t1539).*1.0e-1).*(-1.0./2.0)+dq1.*dq2.*t19.*1.11678e-2;
et17 = dq1.*dq2.*t20.*(7.0./2.5e+2)-dq1.*dq3.*t20.*3.7226e-1-dq1.*dq2.*t23.*(7.0./2.5e+2)-dq1.*dq3.*t22.*1.05e-2+q3.*t3.*t13.*(7.0./1.0e+3)-t3.*t4.*t1303.*5.0e-2+t3.*t9.*t1304.*5.0e-2-(t3.*t4.*t1637)./2.0+(t3.*t9.*t1639)./2.0-dq1.*dq2.*q3.*t19.*(2.1e+1./1.0e+3)+dq1.*dq3.*q3.*t20.*(7.0./1.0e+1);
et18 = dq1.*dq2.*t3.*t8.*1.79512662132e+2-(t2.*t3.*t291.*t1463)./1.0e+2+(t3.*t7.*t291.*t1461)./1.0e+2+dq1.*dq2.*q3.*t3.*t8.*7.4452e-1-dq1.*dq2.*t3.*t8.*t18.*(7.0./1.0e+1);
et19 = t1652+t1324.*t1371.*1.0e-1-t1344.*t1520.*1.0e-1+t1346.*t1542.*1.0e-1-t1322.*t1629.*1.0e-1;
et20 = t1317.*t1635.*1.0e-1;
et21 = t1652+t845.*t1531.*1.0e-1-t1322.*t1618.*1.0e-1+t1317.*t1630.*1.0e-1-t1266.*t1682.*1.0e-1;
et22 = t1273.*(t1263+t1356-t1381-t1539).*1.0e-1;
et23 = t53.*t846.*(-1.0e-1)-t60.*t846.*1.0e-1-t118.*t1323.*1.0e-1+t129.*t1326.*1.0e-1;
et24 = t146.*t1326.*1.0e-1+t178.*t1323.*1.0e-1+t183.*t1323.*1.0e-1-t229.*t1326.*1.0e-1;
et25 = t8.*t9.*t1382.*1.0e-1+t3.*t35.*t1522.*1.0e-1+t3.*t31.*t1543.*1.0e-1;
et26 = t1666+t1327.*t1531.*1.0e-1+t1682.*(t288-t1282).*1.0e-1-t1628.*(t1197-t1340).*1.0e-1+t1634.*(t1258-t1341).*1.0e-1;
et27 = (t297-t1284).*(t1263+t1356-t1381-t1539).*(-1.0e-1);
et28 = t1666+t1324.*t1532.*1.0e-1+t1346.*t1681.*1.0e-1-t1344.*t1687.*1.0e-1-t1619.*(t1197-t1340).*1.0e-1;
et29 = t1631.*(t1258-t1341).*1.0e-1;
et30 = t835.*t846.*(-1.0e-1)+t1042.*t1044.*1.0e-1+t1210.*t1372.*1.0e-1+t1205.*t1384.*1.0e-1;
et31 = t1323.*t1332.*1.0e-1+t1326.*t1334.*1.0e-1;
et32 = (t1804.*(-t1044.*t1045+t1205.*t1322+t1210.*t1317))./2.0+(t1806.*(t845.*t1325-t1266.*t1411+t1273.*t1428))./2.0+(t1805.*((t845.*t1325)./1.0e+1-(t1266.*t1411)./1.0e+1+(t1273.*t1428)./1.0e+1))./2.0-(t1808.*(t1045.*t1324+t1317.*t1346+t1322.*t1344))./2.0;
et33 = (t1801.*(t1044.*t1045.*(-1.0e-1)+t1205.*t1322.*1.0e-1+t1210.*t1317.*1.0e-1))./2.0;
et34 = t1807.*(t1045.*t1324.*1.0e-1+t1317.*t1346.*1.0e-1+t1322.*t1344.*1.0e-1).*(-1.0./2.0)+(t1796.*(t1568+t1324.*t1371-t1344.*t1520+t1346.*t1542-t1322.*t1629+t1317.*t1635))./2.0+(t1783.*(et19+et20))./2.0;
et35 = (t1640.*(t131.*t850+t136.*t850+t144.*t850+t113.*t1046-t185.*t1046-t193.*t1046+t9.*t20.*t25-t9.*t23.*t25-t3.*t32.*t1372-t3.*t28.*t1384+dq4.*t3.*t8.*t21-dq4.*t3.*t8.*t24))./2.0+(t1606.*((t131.*t850)./1.0e+1+(t136.*t850)./1.0e+1+(t144.*t850)./1.0e+1+(t113.*t1046)./1.0e+1-(t185.*t1046)./1.0e+1-(t193.*t1046)./1.0e+1+(t9.*t20.*t25)./1.0e+1-(t9.*t23.*t25)./1.0e+1-(t3.*t32.*t1372)./1.0e+1-(t3.*t28.*t1384)./1.0e+1+(dq4.*t3.*t8.*t21)./1.0e+1-(dq4.*t3.*t8.*t24)./1.0e+1))./2.0-(t1248.*(dq3.*t3-dq2.*t8.*t291))./1.0e+2;
et36 = (t1734.*(t1414-t1491+t1492+t8.*t9.*t1371-t3.*t31.*t1520+t3.*t35.*t1542))./2.0+(t1728.*(t1432-t1500+t1504+(t8.*t9.*t1371)./1.0e+1-(t3.*t31.*t1520)./1.0e+1+(t3.*t35.*t1542)./1.0e+1))./2.0-(t1647.*(t29./1.0e+2-t106./1.0e+2+t3.*t555))./1.0e+2-dq2.*dq3.*3.7226e-1-(t1766.*(t1457+t1577-t1581-t1327.*t1371+t1520.*(t288-t1282)-t1542.*(t297-t1284)))./2.0-(t1765.*(t1480+t1586-t1593-(t1327.*t1371)./1.0e+1+(t1520.*(t288-t1282))./1.0e+1-(t1542.*(t297-t1284))./1.0e+1))./2.0;
et37 = t12.*t19.*(-5.5839e-3)-t12.*t20.*(7.0./5.0e+2)+t12.*t23.*(7.0./5.0e+2)-t4.*t1304.*5.0e-2-t9.*t1303.*5.0e-2-(t4.*t1639)./2.0-(t9.*t1637)./2.0-(t1798.*(t8.*t9.*t846+t3.*t31.*t1323-t3.*t35.*t1326))./2.0;
et38 = t1790.*(t8.*t9.*t846.*1.0e-1+t3.*t31.*t1323.*1.0e-1-t3.*t35.*t1326.*1.0e-1).*(-1.0./2.0)-(t1802.*(t296.*1.0e+2+t1205.*9.1e+1-t2.*t8.*1.56e+2+t6.*t86.*1.0e+2+t6.*t285.*1.0e+2+q3.*t2.*t8.*1.0e+4))./1.0e+10;
et39 = t1803.*(t308.*1.0e+2+t1210.*9.1e+1-t7.*t8.*1.56e+2+t7.*t96.*1.0e+2+t6.*t294.*1.0e+2+q3.*t7.*t8.*1.0e+4).*(-1.0e-10)+(t1728.*(-t1432+t1500-t1504+(t45.*t845)./1.0e+1-(t65.*t845)./1.0e+1+(t1273.*t1372)./1.0e+1+(t1266.*t1384)./1.0e+1))./2.0+(t1734.*(-t1414+t1491-t1492+t45.*t845+t246.*t845+t1273.*t1372+t1266.*t1384))./2.0+(t1776.*(t3.*1.56e+2-t29.*9.1e+1+t74.*1.0e+2-t81.*1.0e+2+t106.*9.1e+1+t300.*1.0e+2-q3.*t3.*1.0e+4))./1.0e+10;
et40 = t1800.*(t850.*t1266-t1046.*t1273+t3.*t9.*t845).*(-1.0./2.0)-(t1799.*((t850.*t1266)./1.0e+1-(t1046.*t1273)./1.0e+1+(t3.*t9.*t845)./1.0e+1))./2.0-(t1796.*(t1568+t845.*t1531-t1322.*t1618+t1317.*t1630-t1266.*t1682+t1273.*(t1263+t1356-t1381-t1539)))./2.0-(t1783.*(et21+et22))./2.0;
et41 = ((t1316.*t1327.*1.0e-1-(t288-t1282).*(t1197-t1340).*1.0e-1+(t297-t1284).*(t1258-t1341).*1.0e-1).*(-t1685-t1732+t1768+t1782.*(t1197-t1340)+t1781.*(t1258-t1341)+t1681.*(t1263+t1356-t1381-t1539)))./2.0;
et42 = ((t1316.*t1327-(t288-t1282).*(t1197-t1340)+(t297-t1284).*(t1258-t1341)).*(-t1701-t1757+t1774+t1782.*(t1197-t1340).*1.0e-1+t1781.*(t1258-t1341).*1.0e-1+t1681.*(t1263+t1356-t1381-t1539).*1.0e-1))./2.0;
et43 = t1770.*(t86./1.0e+2+t285./1.0e+2+t2.*t8.*t555).*(-1.0./1.0e+2)-(t1771.*(t102./1.0e+2+t294./1.0e+2+t7.*t8.*t555))./1.0e+2+(t1737.*(-t53.*t846-t60.*t846+t129.*t1326+t146.*t1326+t178.*t1323+t183.*t1323+t397.*t1323+t446.*t1326+t8.*t9.*t1382+t3.*t35.*t1522+t3.*t31.*t1543))./2.0+(t1668.*(et23+et24+et25))./2.0;
et44 = (t1665+t1687.*(t1197-t1340).*1.0e-1+t1681.*(t1258-t1341).*1.0e-1).*(t1598+t1327.*t1531+t1682.*(t288-t1282)-t1628.*(t1197-t1340)+t1634.*(t1258-t1341)-(t297-t1284).*(t1263+t1356-t1381-t1539)).*(-1.0./2.0)-((t1597+t1687.*(t1197-t1340)+t1681.*(t1258-t1341)).*(et26+et27))./2.0;
et45 = t1640.*(t850.*t1319-t1046.*t1331-t8.*t9.*t836+t3.*t9.*t1041+t3.*t31.*t1373-t3.*t35.*t1385).*(-1.0./2.0)-(t1606.*((t850.*t1319)./1.0e+1-(t1046.*t1331)./1.0e+1-(t8.*t9.*t836)./1.0e+1+(t3.*t9.*t1041)./1.0e+1+(t3.*t31.*t1373)./1.0e+1-(t3.*t35.*t1385)./1.0e+1))./2.0-(t1772.*(t1437-t1525+t1527+t845.*t1382-t1273.*t1522-t1266.*t1543))./2.0+(t1772.*(t1437-t1525+t1527-t1044.*t1371-t1205.*t1520+t1210.*t1542))./2.0+(t1766.*(t1457+t1577-t1581-t845.*t1532-t1266.*t1687+t1273.*t1681))./2.0;
et46 = (t1765.*(t1480+t1586-t1593-(t845.*t1532)./1.0e+1-(t1266.*t1687)./1.0e+1+(t1273.*t1681)./1.0e+1))./2.0-(t1754.*(t1521-t1620+t1622+t845.*t1382.*1.0e-1-t1273.*t1522.*1.0e-1-t1266.*t1543.*1.0e-1))./2.0;
et47 = (t1754.*(t1521-t1620+t1622-t1044.*t1371.*1.0e-1-t1205.*t1520.*1.0e-1+t1210.*t1542.*1.0e-1))./2.0;
et48 = ((t1665+t1687.*(t1197-t1340).*1.0e-1+t1681.*(t1258-t1341).*1.0e-1).*(t1598+t1324.*t1532+t1346.*t1681-t1344.*t1687-t1619.*(t1197-t1340)+t1631.*(t1258-t1341)))./2.0+((t1597+t1687.*(t1197-t1340)+t1681.*(t1258-t1341)).*(et28+et29))./2.0+(t1780.*(-t3.*t28.*t850+t3.*t32.*t1046+t3.*t4.*t8.*t9))./2.0;
et49 = (t1777.*(t3.*t28.*t850.*(-1.0./1.0e+1)+(t3.*t32.*t1046)./1.0e+1+(t3.*t4.*t8.*t9)./1.0e+1))./2.0-(t1737.*(-t835.*t846+t1042.*t1044+t1210.*t1372+t1205.*t1384+t1323.*t1332+t1326.*t1334))./2.0-(t1668.*(et30+et31))./2.0-(t1374.*(t2.*t26+t2.*t847-dq1.*t7.*t8.*t291))./1.0e+2+(t1376.*(t7.*t26+t7.*t847+dq1.*t2.*t8.*t291))./1.0e+2+dq2.*dq3.*q3.*(7.0./1.0e+1)+dq4.*t4.*t595.*5.0e-2;
et50 = dq4.*t9.*t851.*(-5.0e-2)+(dq3.*t3.*t1248)./1.0e+2+(dq4.*t4.*t1511)./2.0-(dq4.*t9.*t1513)./2.0+q3.*t12.*t19.*1.05e-2-t3.*t8.*t12.*8.9756331066e+1+(t2.*t26.*t1374)./1.0e+2-(t7.*t26.*t1376)./1.0e+2+(t2.*t847.*t1374)./1.0e+2-(t7.*t847.*t1376)./1.0e+2+(t3.*t291.*(t70-t1137))./1.0e+2;
et51 = dq1.*t4.*t8.*t595.*5.0e-2-dq1.*t8.*t9.*t851.*5.0e-2+(dq1.*t4.*t8.*t1511)./2.0-(dq1.*t8.*t9.*t1513)./2.0-(dq2.*t8.*t291.*t1248)./1.0e+2-q3.*t3.*t8.*t12.*3.7226e-1+t3.*t8.*t12.*t18.*(7.0./2.0e+1)+(t2.*t8.*t291.*t1461)./1.0e+2+(t7.*t8.*t291.*t1463)./1.0e+2-(dq1.*t2.*t8.*t291.*t1376)./1.0e+2-(dq1.*t7.*t8.*t291.*t1374)./1.0e+2;
et52 = t13.*1.8613e-1-q3.*t13.*(7.0./2.0e+1)+t12.*t20.*1.8613e-1+t12.*t22.*5.25e-3+(t38.*t1376)./1.0e+2+(t47.*t1374)./1.0e+2+(t48.*t1374)./1.0e+2-(t63.*t1376)./1.0e+2-(t8.*t1647)./1.0e+2-(t38.*t1676)./1.0e+2+(t47.*t1675)./1.0e+2+(t48.*t1675)./1.0e+2+(t63.*t1676)./1.0e+2-(t8.*t1776)./1.0e+6-(t38.*t1778)./1.0e+6+(t47.*t1779)./1.0e+6+(t48.*t1779)./1.0e+6+(t63.*t1778)./1.0e+6-(t834.*t1374)./1.0e+2;
et53 = t1040.*t1376.*(-1.0./1.0e+2)-(t834.*t1675)./1.0e+2-(t834.*t1779)./1.0e+6+(t1040.*t1676)./1.0e+2+(t8.*(t70-t1137))./1.0e+2+(t1778.*(t38.*1.0e+4-t63.*1.0e+4))./1.0e+10-q3.*t12.*t20.*(7.0./2.0e+1)-(t2.*t3.*t1461)./1.0e+2-(t3.*t7.*t1463)./1.0e+2+(t2.*t3.*t1770)./1.0e+2+(t3.*t7.*t1771)./1.0e+2+(t2.*t3.*t1802)./1.0e+6+(t3.*t7.*t1803)./1.0e+6;
et54 = t1597+t1687.*(t1197-t1340)+t1681.*(t1258-t1341);
et55 = (-t1621+t1708-t1272.*t1532.*1.0e-1+t1378.*t1681.*1.0e-1+t1377.*t1687.*1.0e-1+t1660.*(t1197-t1340).*1.0e-1)./2.0;
et56 = t1615+t1625+t160.*t1045.*1.0e-1+t169.*t1045.*1.0e-1-t233.*t1045.*1.0e-1+t1211.*t1520.*1.0e-1;
et57 = t1275.*t1542.*1.0e-1+t9.*t33.*t1371.*1.0e-1;
et58 = t1563+t1570+t54.*t846.*1.0e-1+t59.*t846.*1.0e-1-t849.*t1522.*1.0e-1+t1047.*t1543.*1.0e-1;
et59 = t3.*t4.*t1382.*1.0e-1;
et60 = (t1606.*((t850.*t1384)./5.0-(t1046.*t1372)./5.0-(dq2.*t3.*t8.*t24)./5.0+(dq4.*t4.*t9.*t20)./5.0))./2.0+(t1640.*(t850.*t1384.*2.0-t1046.*t1372.*2.0-dq2.*t3.*t8.*t24.*2.0+dq4.*t4.*t9.*t20.*2.0))./2.0+(t1808.*(t1045.*t1272-t1317.*t1378+t1322.*t1377))./2.0;
et61 = (t1807.*(t1045.*t1272.*1.0e-1-t1317.*t1378.*1.0e-1+t1322.*t1377.*1.0e-1))./2.0-(t1734.*(t1493+t1498-t1208.*t1384+t1271.*t1372+t8.*t24.*t43.*2.0+dq5.*t10.*t20.*t24-dq4.*t4.*t5.*t9.*t20.*2.0))./2.0;
et62 = t1728.*(t1505+t1507-(t1208.*t1384)./1.0e+1+(t1271.*t1372)./1.0e+1+(t8.*t24.*t43)./5.0+(dq5.*t10.*t20.*t24)./1.0e+1-(dq4.*t4.*t5.*t9.*t20)./5.0).*(-1.0./2.0)+((t1665+t1687.*(t1197-t1340).*1.0e-1+t1681.*(t1258-t1341).*1.0e-1).*(-t1526+t1689-t1272.*t1532+t1378.*t1681+t1377.*t1687+t1660.*(t1197-t1340)))./2.0+et54.*et55;
et63 = (t1734.*(t1493+t1498+t849.*t1542+t1047.*t1520+t3.*t9.*t1333-t3.*t4.*t1371))./2.0+(t1728.*(t1505+t1507+(t849.*t1542)./1.0e+1+(t1047.*t1520)./1.0e+1+(t3.*t9.*t1333)./1.0e+1-(t3.*t4.*t1371)./1.0e+1))./2.0+(t1776.*(t93.*-1.0e+2+t299.*1.0e+2+t9.*t33.*9.1e+1))./1.0e+10+(t1777.*(t1136./1.0e+1+t1246./1.0e+1+(t20.*t24)./1.0e+1))./2.0+(t1802.*(t1211.*9.1e+1+t11.*t35.*1.0e+2-t11.*t84.*1.0e+2+t6.*t104.*1.0e+2+t31.*t110.*1.0e+2))./1.0e+10+(t1772.*(t1519+t1541+t160.*t1045+t169.*t1045+t450.*t1045+t1211.*t1520+t1275.*t1542+t9.*t33.*t1371))./2.0;
et64 = t1766.*(t1582+t1587+t123.*t1325-t196.*t1325-t215.*t1325+t1208.*t1687+t1271.*t1681+t9.*t29.*t1532).*(-1.0./2.0)-(t1765.*(t1594+t1599+(t123.*t1325)./1.0e+1-(t196.*t1325)./1.0e+1-(t215.*t1325)./1.0e+1+(t1208.*t1687)./1.0e+1+(t1271.*t1681)./1.0e+1+(t9.*t29.*t1532)./1.0e+1))./2.0+(t1754.*(et56+et57))./2.0-(t160.*t1495)./1.0e+4-(t169.*t1495)./1.0e+4+(t233.*t1495)./1.0e+4-(t1796.*(t1506+t1678+t1679-t1208.*t1682-t1271.*(t1263+t1356-t1381-t1539)+t9.*t29.*t1531))./2.0;
et65 = t1783.*(t1605+t1695+t1697-t1208.*t1682.*1.0e-1-t1271.*(t1263+t1356-t1381-t1539).*1.0e-1+t9.*t29.*t1531.*1.0e-1).*(-1.0./2.0)+(t1780.*(t1136+t1246+t20.*t24))./2.0+(t1796.*(t1506+t1678+t1679-t1272.*t1371+t1377.*t1520+t1378.*t1542))./2.0;
et66 = (t1783.*(t1605+t1695+t1697-t1272.*t1371.*1.0e-1+t1377.*t1520.*1.0e-1+t1378.*t1542.*1.0e-1))./2.0-(t1800.*(t850.*t1208+t1046.*t1271+t5.*t20.*t24))./2.0-(t1799.*((t850.*t1208)./1.0e+1+(t1046.*t1271)./1.0e+1+(t5.*t20.*t24)./1.0e+1))./2.0;
et67 = (t1798.*(t849.*t1326+t1047.*t1323+t3.*t4.*t846))./2.0+(t1804.*(-t1211.*t1322+t1275.*t1317+t9.*t33.*t1045))./2.0-(t1806.*(t1208.*t1411+t1271.*t1428-t9.*t29.*t1325))./2.0-(t1805.*((t1208.*t1411)./1.0e+1+(t1271.*t1428)./1.0e+1-(t9.*t29.*t1325)./1.0e+1))./2.0;
et68 = (t1790.*(t849.*t1326.*1.0e-1+t1047.*t1323.*1.0e-1+t3.*t4.*t846.*1.0e-1))./2.0;
et69 = (t1801.*(t1211.*t1322.*(-1.0e-1)+t1275.*t1317.*1.0e-1+t9.*t33.*t1045.*1.0e-1))./2.0;
et70 = ((t1209.*t1316.*(-1.0e-1)+(t1197-t1340).*(t1253-t1286).*1.0e-1+(t1191-t1307).*(t1258-t1341).*1.0e-1).*(-t1685-t1732+t1768+t1782.*(t1197-t1340)+t1781.*(t1258-t1341)+t1681.*(t1263+t1356-t1381-t1539)))./2.0;
et71 = ((-t1209.*t1316+(t1197-t1340).*(t1253-t1286)+(t1191-t1307).*(t1258-t1341)).*(-t1701-t1757+t1774+t1782.*(t1197-t1340).*1.0e-1+t1781.*(t1258-t1341).*1.0e-1+t1681.*(t1263+t1356-t1381-t1539).*1.0e-1))./2.0;
et72 = (t1766.*(t1582+t1587-t1209.*t1371-t1325.*t1333+t1542.*(t1191-t1307)+t1520.*(t1253-t1286)))./2.0+(t1765.*(t1594+t1599-(t1209.*t1371)./1.0e+1-(t1325.*t1333)./1.0e+1+(t1542.*(t1191-t1307))./1.0e+1+(t1520.*(t1253-t1286))./1.0e+1))./2.0-(t1737.*(t1447+t1459-t836.*t846-t1211.*t1384+t1275.*t1372-t9.*t33.*t1042))./2.0+(t1772.*(t1516+t1528-t1045.*t1335+t1208.*t1543-t1271.*t1522-t9.*t29.*t1382))./2.0;
et73 = t1668.*(t1561+t1566-t836.*t846.*1.0e-1-t1211.*t1384.*1.0e-1+t1275.*t1372.*1.0e-1-t9.*t33.*t1042.*1.0e-1).*(-1.0./2.0);
et74 = (t1754.*(t1611+t1623-t1045.*t1335.*1.0e-1+t1208.*t1543.*1.0e-1-t1271.*t1522.*1.0e-1-t9.*t29.*t1382.*1.0e-1))./2.0;
et75 = (t1495.*(t160./1.0e+2+t169./1.0e+2-t233./1.0e+2))./1.0e+2+(t1640.*(t849.*t1385-t850.*t1384+t1046.*t1372+t1047.*t1373-t3.*t4.*t836-t3.*t9.*t1042))./2.0+(t1606.*((t849.*t1385)./1.0e+1-(t850.*t1384)./1.0e+1+(t1046.*t1372)./1.0e+1+(t1047.*t1373)./1.0e+1-(t3.*t4.*t836)./1.0e+1-(t3.*t9.*t1042)./1.0e+1))./2.0-(t1771.*(t88./1.0e+2-t316./1.0e+2))./1.0e+2+(t1770.*(t104./1.0e+2+t305./1.0e+2))./1.0e+2-(t1737.*(t1455+t1470+t54.*t846+t59.*t846-t849.*t1522+t1047.*t1543+t3.*t4.*t1382))./2.0-(t1668.*(et58+et59))./2.0;
et76 = t1803.*(t88.*9.1e+1-t316.*9.1e+1+t11.*t31.*1.0e+2+t6.*t88.*1.0e+2+t11.*t99.*1.0e+2-t35.*t110.*1.0e+2).*(-1.0e-10)+((t1665+t1687.*(t1197-t1340).*1.0e-1+t1681.*(t1258-t1341).*1.0e-1).*(t1526+t1688-t1689+t1209.*t1531+t1682.*(t1253-t1286)+(t1191-t1307).*(t1263+t1356-t1381-t1539)))./2.0;
et77 = ((t1597+t1687.*(t1197-t1340)+t1681.*(t1258-t1341)).*(t1621+t1705-t1708+t1209.*t1531.*1.0e-1+t1682.*(t1253-t1286).*1.0e-1+(t1191-t1307).*(t1263+t1356-t1381-t1539).*1.0e-1))./2.0+(t9.*t33.*t1647)./1.0e+4;
et78 = t1610-t11.*t1692.*1.0e-1-t1274.*t1531.*1.0e-1-t1347.*(t1197-t1340).*1.0e-1+t1337.*(t1258-t1341).*1.0e-1;
et79 = t1538.*(t1197-t1340).*1.0e-1+t1553.*(t1258-t1341).*1.0e-1+t11.*t1317.*(t1263+t1356-t1381-t1539).*1.0e-1;
et80 = t1601+t846.*t1531.*1.0e-1-t1322.*t1607.*1.0e-1+t1323.*t1682.*1.0e-1-t1317.*(t1338-t1551).*1.0e-1;
et81 = t1326.*(t1263+t1356-t1381-t1539).*1.0e-1;
et82 = t1601+t1267.*t1371.*1.0e-1-t1322.*t1537.*2.0e-1+t1317.*t1551.*2.0e-1-dq6.*t11.*t1329.*1.0e-1;
et83 = dq6.*t11.*t1336.*(-1.0e-1);
et84 = t846.*t1382.*1.0e-1+t1045.*t1371.*1.0e-1-t1322.*t1520.*1.0e-1-t1326.*t1522.*1.0e-1;
et85 = t1317.*t1542.*1.0e-1+t1323.*t1543.*1.0e-1;
et86 = t1597+t1687.*(t1197-t1340)+t1681.*(t1258-t1341);
et87 = (t1610-t6.*t1696.*1.0e-1+t6.*t1716+t1267.*t1532.*1.0e-1+t1609.*(t1258-t1341).*1.0e-1-(t1197-t1340).*(t1347-t1538).*1.0e-1)./2.0;
et88 = t1808.*(t6.*t1329+t6.*t1336+t1045.*t1267).*(-1.0./2.0)-(t1807.*(t6.*t1329.*1.0e-1+t6.*t1336.*1.0e-1+t1045.*t1267.*1.0e-1))./2.0-(t1737.*(-t1042.*t1045+t1317.*t1372+t1322.*t1384))./2.0+(t1806.*(t846.*t1325+t1323.*t1411+t1326.*t1428))./2.0;
et89 = (t1805.*((t846.*t1325)./1.0e+1+(t1323.*t1411)./1.0e+1+(t1326.*t1428)./1.0e+1))./2.0+(t1772.*(t1045.*t1371.*2.0-t1322.*t1520.*2.0+t1317.*t1542.*2.0))./2.0-(t1668.*(t1042.*t1045.*(-1.0e-1)+t1317.*t1372.*1.0e-1+t1322.*t1384.*1.0e-1))./2.0;
et90 = (t1754.*(t1045.*t1371.*2.0e-1-t1322.*t1520.*2.0e-1+t1317.*t1542.*2.0e-1))./2.0;
et91 = (t1274.*t1316.*1.0e-1-t11.*t1322.*(t1197-t1340).*1.0e-1+t11.*t1317.*(t1258-t1341).*1.0e-1).*(-t1685-t1732+t1768+t1782.*(t1197-t1340)+t1781.*(t1258-t1341)+t1681.*(t1263+t1356-t1381-t1539)).*(-1.0./2.0);
et92 = (t1274.*t1316-t11.*t1322.*(t1197-t1340)+t11.*t1317.*(t1258-t1341)).*(-t1701-t1757+t1774+t1782.*(t1197-t1340).*1.0e-1+t1781.*(t1258-t1341).*1.0e-1+t1681.*(t1263+t1356-t1381-t1539).*1.0e-1).*(-1.0./2.0);
et93 = t1734.*(t1413-t1444+t1458+t1571+t1579-t45.*t846+t65.*t846).*(-1.0./2.0)-(t1766.*(t1456+t1646+t1648+t1274.*t1371-t1322.*t1538+t1317.*t1553))./2.0+(t1766.*(t1456+t1646+t1648-t846.*t1532+t1326.*t1681+t1323.*t1687))./2.0-(t1765.*(t1479+t1653+t1654+(t1274.*t1371)./1.0e+1-(t1322.*t1538)./1.0e+1+(t1317.*t1553)./1.0e+1))./2.0+(t1765.*(t1479+t1653+t1654-(t846.*t1532)./1.0e+1+(t1326.*t1681)./1.0e+1+(t1323.*t1687)./1.0e+1))./2.0+(t1800.*(t850.*t1323+t1046.*t1326-t3.*t9.*t846))./2.0+(t1799.*((t850.*t1323)./1.0e+1+(t1046.*t1326)./1.0e+1-(t3.*t9.*t846)./1.0e+1))./2.0;
et94 = (t1776.*(t36.*9.1e+1-t79.*9.1e+1+t110.*1.0e+2-t284.*1.0e+2))./1.0e+10-(t1802.*(t85.*9.1e+1-t105.*9.1e+1+t286.*9.1e+1+t6.*t85.*1.0e+2-t6.*t105.*1.0e+2+t28.*t96.*1.0e+2))./1.0e+10+(t1804.*(t1245+t1329+t1336))./2.0+(t1734.*(t1413+t1571+t1579))./2.0+(t1728.*(t1431+t1580+t1585))./2.0;
et95 = (t1665+t1687.*(t1197-t1340).*1.0e-1+t1681.*(t1258-t1341).*1.0e-1).*(t1515-t11.*t1692-t1274.*t1531+t1364.*(t1197-t1340)+t1337.*(t1258-t1341)+t1538.*(t1197-t1340)+t1553.*(t1258-t1341)+t11.*t1317.*(t1263+t1356-t1381-t1539)).*(-1.0./2.0)-((t1597+t1687.*(t1197-t1340)+t1681.*(t1258-t1341)).*(et78+et79))./2.0;
et96 = t1770.*(t85./1.0e+2-t105./1.0e+2+t286./1.0e+2).*(-1.0./1.0e+2)-(t1771.*(t89./1.0e+2+t101./1.0e+2+t295./1.0e+2))./1.0e+2+(t1801.*(t1245.*1.0e-1+t1329.*1.0e-1+t1336.*1.0e-1))./2.0;
et97 = t1796.*(t1496+t846.*t1531-t1322.*t1607+t1323.*t1682-t1317.*(t1338-t1551)+t1326.*(t1263+t1356-t1381-t1539)).*(-1.0./2.0)-(t1783.*(et80+et81))./2.0-(t1728.*(t1431-t1444./1.0e+1+t1458./1.0e+1+t1580+t1585-(t45.*t846)./1.0e+1+(t65.*t846)./1.0e+1))./2.0+(t1796.*(t1496+t1267.*t1371-t1322.*t1537.*2.0+t1317.*t1551.*2.0-dq6.*t11.*t1329-dq6.*t11.*t1336))./2.0+(t1783.*(et82+et83))./2.0+(t1647.*(t36./1.0e+2-t79./1.0e+2))./1.0e+2-(t1803.*(t1317.*9.1e+1+t6.*t89.*1.0e+2+t6.*t101.*1.0e+2+t32.*t96.*1.0e+2))./1.0e+10;
et98 = t1772.*(t846.*t1382+t1045.*t1371-t1322.*t1520-t1326.*t1522+t1317.*t1542+t1323.*t1543).*(-1.0./2.0)-(t1754.*(et84+et85))./2.0+((t1665+t1687.*(t1197-t1340).*1.0e-1+t1681.*(t1258-t1341).*1.0e-1).*(t1515+t6.*t1691+t6.*t1698+t1267.*t1532+t1609.*(t1258-t1341)-(t1197-t1340).*(t1347-t1538)))./2.0+et86.*et87;
et99 = t1316.*t1531.*(-1.0e-1)-t1325.*t1532.*1.0e-1+t1411.*t1687.*1.0e-1+t1428.*t1681.*1.0e-1;
et100 = t1682.*(t1197-t1340).*1.0e-1+(t1258-t1341).*(t1263+t1356-t1381-t1539).*1.0e-1;
et101 = t1808.*(t1045.*t1325+t1322.*t1411-t1317.*t1428).*(-1.0./2.0)-(t1807.*(t1045.*t1325.*1.0e-1+t1322.*t1411.*1.0e-1-t1317.*t1428.*1.0e-1))./2.0;
et102 = (t1783.*(t1445.*1.0e-1-t1643.*1.0e-1-t1650.*1.0e-1+t1656+t1716+t1726))./2.0;
et103 = (t1665+t1687.*(t1197-t1340).*1.0e-1+t1681.*(t1258-t1341).*1.0e-1).*(-t1316.*t1531-t1325.*t1532+t1411.*t1687+t1428.*t1681+t1682.*(t1197-t1340)+(t1258-t1341).*(t1263+t1356-t1381-t1539)).*(-1.0./2.0)-((t1597+t1687.*(t1197-t1340)+t1681.*(t1258-t1341)).*(et99+et100))./2.0;
et104 = ((t1316.*t1531.*-2.0+t1682.*(t1197-t1340).*2.0+(t1258-t1341).*(t1263+t1356-t1381-t1539).*2.0).*(t1665+t1687.*(t1197-t1340).*1.0e-1+t1681.*(t1258-t1341).*1.0e-1))./2.0;
et105 = ((t1316.*t1531.*(-2.0e-1)+t1682.*(t1197-t1340).*2.0e-1+(t1258-t1341).*(t1263+t1356-t1381-t1539).*2.0e-1).*(t1597+t1687.*(t1197-t1340)+t1681.*(t1258-t1341)))./2.0;
et106 = ((t1328+t1434+t1435).*(-t1701-t1757+t1774+t1782.*(t1197-t1340).*1.0e-1+t1781.*(t1258-t1341).*1.0e-1+t1681.*(t1263+t1356-t1381-t1539).*1.0e-1))./2.0;
et107 = ((t1328.*1.0e-1+t1434.*1.0e-1+t1435.*1.0e-1).*(-t1685-t1732+t1768+t1782.*(t1197-t1340)+t1781.*(t1258-t1341)+t1681.*(t1263+t1356-t1381-t1539)))./2.0+(t1766.*(t1316.*t1371+t1520.*(t1197-t1340)+t1542.*(t1258-t1341)))./2.0;
et108 = (t1765.*((t1316.*t1371)./1.0e+1+(t1520.*(t1197-t1340))./1.0e+1+(t1542.*(t1258-t1341))./1.0e+1))./2.0-(t1796.*(t1573+t1691+t1698))./2.0-(t1783.*(t1656+t1716+t1726))./2.0-(t1802.*(t6.*t32.*1.0e+2+t11.*t73.*1.0e+2+t11.*t77.*1.0e+2-t28.*t75.*1.0e+2+t6.*t98.*1.0e+2))./1.0e+10+(t1803.*(t6.*t28.*1.0e+2-t6.*t71.*1.0e+2-t11.*t87.*1.0e+2+t32.*t75.*1.0e+2+t11.*t103.*1.0e+2))./1.0e+10+(t1796.*(t1445+t1573-t1643-t1650+t1691+t1698))./2.0;
et109 = (t1776.*(t94.*-1.0e+2+t109.*1.0e+2+t298.*1.0e+2))./1.0e+10;
C = [et3+et4+et5+et6+et7+et8+et9+et10+et11+et12+et13+et14+et15+et16+et17+et18;et32+et33+et34+et35+et36+et37+et38+et39+et40+et41+et42+et43+et44+et45+et46+et47+et48+et49+et50+et51;et52+et53;et60+et61+et62+et63+et64+et65+et66+et67+et68+et69+et70+et71+et72+et73+et74+et75+et76+et77;et88+et89+et90+et91+et92+et93+et94+et95+et96+et97+et98;et101+et102+et103+et104+et105+et106+et107+et108+et109];
end
